simulink model "deng_feng_unpack"  (R2016b)
(part 2 of 28)

      | port_label('input', 1, 'd');
      | port_label('output', 1, 'q');
      | disp(['Z^-', num2str(latency)]);
  pipeline249 : Subsystem  AncestorBlock=casper_library_delays/pipeline  mask(pipeline){latency=2}
      mask help:
      | An explicitly laid-out delay line to avoid mapping to SRL16s
      | for use in pipelining to help achieve timing closure.
      mask init:
      | pipeline_init(gcb,'latency',latency);
      settings: AttributesFormatString=Latency = %<latency>
      mask Display:
      | port_label('input', 1, 'd');
      | port_label('output', 1, 'q');
      | disp(['Z^-', num2str(latency)]);
  pipeline251 : Subsystem  AncestorBlock=casper_library_delays/pipeline  mask(pipeline){latency=2}
      mask help:
      | An explicitly laid-out delay line to avoid mapping to SRL16s
      | for use in pipelining to help achieve timing closure.
      mask init:
      | pipeline_init(gcb,'latency',latency);
      settings: AttributesFormatString=Latency = %<latency>
      mask Display:
      | port_label('input', 1, 'd');
      | port_label('output', 1, 'q');
      | disp(['Z^-', num2str(latency)]);
  pipeline252 : Subsystem  AncestorBlock=casper_library_delays/pipeline  mask(pipeline){latency=2}
      mask help:
      | An explicitly laid-out delay line to avoid mapping to SRL16s
      | for use in pipelining to help achieve timing closure.
      mask init:
      | pipeline_init(gcb,'latency',latency);
      settings: AttributesFormatString=Latency = %<latency>
      mask Display:
      | port_label('input', 1, 'd');
      | port_label('output', 1, 'q');
      | disp(['Z^-', num2str(latency)]);
  pipeline257 : Subsystem  AncestorBlock=casper_library_delays/pipeline  mask(pipeline){latency=2}
      mask help:
      | An explicitly laid-out delay line to avoid mapping to SRL16s
      | for use in pipelining to help achieve timing closure.
      mask init:
      | pipeline_init(gcb,'latency',latency);
      settings: AttributesFormatString=Latency = %<latency>
      mask Display:
      | port_label('input', 1, 'd');
      | port_label('output', 1, 'q');
      | disp(['Z^-', num2str(latency)]);
  pipeline258 : Subsystem  AncestorBlock=casper_library_delays/pipeline  mask(pipeline){latency=2}
      mask help:
      | An explicitly laid-out delay line to avoid mapping to SRL16s
      | for use in pipelining to help achieve timing closure.
      mask init:
      | pipeline_init(gcb,'latency',latency);
      settings: AttributesFormatString=Latency = %<latency>
      mask Display:
      | port_label('input', 1, 'd');
      | port_label('output', 1, 'q');
      | disp(['Z^-', num2str(latency)]);
  pipeline263 : Subsystem  AncestorBlock=casper_library_delays/pipeline  mask(pipeline){latency=2}
      mask help:
      | An explicitly laid-out delay line to avoid mapping to SRL16s
      | for use in pipelining to help achieve timing closure.
      mask init:
      | pipeline_init(gcb,'latency',latency);
      settings: AttributesFormatString=Latency = %<latency>
      mask Display:
      | port_label('input', 1, 'd');
      | port_label('output', 1, 'q');
      | disp(['Z^-', num2str(latency)]);
  pipeline264 : Subsystem  AncestorBlock=casper_library_delays/pipeline  mask(pipeline){latency=2}
      mask help:
      | An explicitly laid-out delay line to avoid mapping to SRL16s
      | for use in pipelining to help achieve timing closure.
      mask init:
      | pipeline_init(gcb,'latency',latency);
      settings: AttributesFormatString=Latency = %<latency>
      mask Display:
      | port_label('input', 1, 'd');
      | port_label('output', 1, 'q');
      | disp(['Z^-', num2str(latency)]);
  pipeline268 : Subsystem  AncestorBlock=casper_library_delays/pipeline  mask(pipeline){latency=2}
      mask help:
      | An explicitly laid-out delay line to avoid mapping to SRL16s
      | for use in pipelining to help achieve timing closure.
      mask init:
      | pipeline_init(gcb,'latency',latency);
      settings: AttributesFormatString=Latency = %<latency>
      mask Display:
      | port_label('input', 1, 'd');
      | port_label('output', 1, 'q');
      | disp(['Z^-', num2str(latency)]);
  pipeline270 : Subsystem  AncestorBlock=casper_library_delays/pipeline  mask(pipeline){latency=1}
      mask help:
      | An explicitly laid-out delay line to avoid mapping to SRL16s
      | for use in pipelining to help achieve timing closure.
      mask init:
      | pipeline_init(gcb,'latency',latency);
      settings: AttributesFormatString=Latency = %<latency>
      mask Display:
      | port_label('input', 1, 'd');
      | port_label('output', 1, 'q');
      | disp(['Z^-', num2str(latency)]);
  pipeline271 : Subsystem  AncestorBlock=casper_library_delays/pipeline  mask(pipeline){latency=2}
      mask help:
      | An explicitly laid-out delay line to avoid mapping to SRL16s
      | for use in pipelining to help achieve timing closure.
      mask init:
      | pipeline_init(gcb,'latency',latency);
      settings: AttributesFormatString=Latency = %<latency>
      mask Display:
      | port_label('input', 1, 'd');
      | port_label('output', 1, 'q');
      | disp(['Z^-', num2str(latency)]);
  pipeline272 : Subsystem  AncestorBlock=casper_library_delays/pipeline  mask(pipeline){latency=2}
      mask help:
      | An explicitly laid-out delay line to avoid mapping to SRL16s
      | for use in pipelining to help achieve timing closure.
      mask init:
      | pipeline_init(gcb,'latency',latency);
      settings: AttributesFormatString=Latency = %<latency>
      mask Display:
      | port_label('input', 1, 'd');
      | port_label('output', 1, 'q');
      | disp(['Z^-', num2str(latency)]);
  pipeline273 : Subsystem  AncestorBlock=casper_library_delays/pipeline  mask(pipeline){latency=2}
      mask help:
      | An explicitly laid-out delay line to avoid mapping to SRL16s
      | for use in pipelining to help achieve timing closure.
      mask init:
      | pipeline_init(gcb,'latency',latency);
      settings: AttributesFormatString=Latency = %<latency>
      mask Display:
      | port_label('input', 1, 'd');
      | port_label('output', 1, 'q');
      | disp(['Z^-', num2str(latency)]);
  pipeline274 : Subsystem  AncestorBlock=casper_library_delays/pipeline  mask(pipeline){latency=2}
      mask help:
      | An explicitly laid-out delay line to avoid mapping to SRL16s
      | for use in pipelining to help achieve timing closure.
      mask init:
      | pipeline_init(gcb,'latency',latency);
      settings: AttributesFormatString=Latency = %<latency>
      mask Display:
      | port_label('input', 1, 'd');
      | port_label('output', 1, 'q');
      | disp(['Z^-', num2str(latency)]);
  pipeline275 : Subsystem  AncestorBlock=casper_library_delays/pipeline  mask(pipeline){latency=2}
      mask help:
      | An explicitly laid-out delay line to avoid mapping to SRL16s
      | for use in pipelining to help achieve timing closure.
      mask init:
      | pipeline_init(gcb,'latency',latency);
      settings: AttributesFormatString=Latency = %<latency>
      mask Display:
      | port_label('input', 1, 'd');
      | port_label('output', 1, 'q');
      | disp(['Z^-', num2str(latency)]);
  pipeline276 : Subsystem  AncestorBlock=casper_library_delays/pipeline  mask(pipeline){latency=2}
      mask help:
      | An explicitly laid-out delay line to avoid mapping to SRL16s
      | for use in pipelining to help achieve timing closure.
      mask init:
      | pipeline_init(gcb,'latency',latency);
      settings: AttributesFormatString=Latency = %<latency>
      mask Display:
      | port_label('input', 1, 'd');
      | port_label('output', 1, 'q');
      | disp(['Z^-', num2str(latency)]);
  pipeline277 : Subsystem  AncestorBlock=casper_library_delays/pipeline  mask(pipeline){latency=2}
      mask help:
      | An explicitly laid-out delay line to avoid mapping to SRL16s
      | for use in pipelining to help achieve timing closure.
      mask init:
      | pipeline_init(gcb,'latency',latency);
      settings: AttributesFormatString=Latency = %<latency>
      mask Display:
      | port_label('input', 1, 'd');
      | port_label('output', 1, 'q');
      | disp(['Z^-', num2str(latency)]);
  pipeline278 : Subsystem  AncestorBlock=casper_library_delays/pipeline  mask(pipeline){latency=2}
      mask help:
      | An explicitly laid-out delay line to avoid mapping to SRL16s
      | for use in pipelining to help achieve timing closure.
      mask init:
      | pipeline_init(gcb,'latency',latency);
      settings: AttributesFormatString=Latency = %<latency>
      mask Display:
      | port_label('input', 1, 'd');
      | port_label('output', 1, 'q');
      | disp(['Z^-', num2str(latency)]);
  pipeline285 : Subsystem  AncestorBlock=casper_library_delays/pipeline  mask(pipeline){latency=2}
      mask help:
      | An explicitly laid-out delay line to avoid mapping to SRL16s
      | for use in pipelining to help achieve timing closure.
      mask init:
      | pipeline_init(gcb,'latency',latency);
      settings: AttributesFormatString=Latency = %<latency>
      mask Display:
      | port_label('input', 1, 'd');
      | port_label('output', 1, 'q');
      | disp(['Z^-', num2str(latency)]);
  pipeline286 : Subsystem  AncestorBlock=casper_library_delays/pipeline  mask(pipeline){latency=2}
      mask help:
      | An explicitly laid-out delay line to avoid mapping to SRL16s
      | for use in pipelining to help achieve timing closure.
      mask init:
      | pipeline_init(gcb,'latency',latency);
      settings: AttributesFormatString=Latency = %<latency>
      mask Display:
      | port_label('input', 1, 'd');
      | port_label('output', 1, 'q');
      | disp(['Z^-', num2str(latency)]);
  pipeline287 : Subsystem  AncestorBlock=casper_library_delays/pipeline  mask(pipeline){latency=2}
      mask help:
      | An explicitly laid-out delay line to avoid mapping to SRL16s
      | for use in pipelining to help achieve timing closure.
      mask init:
      | pipeline_init(gcb,'latency',latency);
      settings: AttributesFormatString=Latency = %<latency>
      mask Display:
      | port_label('input', 1, 'd');
      | port_label('output', 1, 'q');
      | disp(['Z^-', num2str(latency)]);
  pipeline288 : Subsystem  AncestorBlock=casper_library_delays/pipeline  mask(pipeline){latency=2}
      mask help:
      | An explicitly laid-out delay line to avoid mapping to SRL16s
      | for use in pipelining to help achieve timing closure.
      mask init:
      | pipeline_init(gcb,'latency',latency);
      settings: AttributesFormatString=Latency = %<latency>
      mask Display:
      | port_label('input', 1, 'd');
      | port_label('output', 1, 'q');
      | disp(['Z^-', num2str(latency)]);
  pipeline289 : Subsystem  AncestorBlock=casper_library_delays/pipeline  mask(pipeline){latency=2}
      mask help:
      | An explicitly laid-out delay line to avoid mapping to SRL16s
      | for use in pipelining to help achieve timing closure.
      mask init:
      | pipeline_init(gcb,'latency',latency);
      settings: AttributesFormatString=Latency = %<latency>
      mask Display:
      | port_label('input', 1, 'd');
      | port_label('output', 1, 'q');
      | disp(['Z^-', num2str(latency)]);
  pipeline290 : Subsystem  AncestorBlock=casper_library_delays/pipeline  mask(pipeline){latency=2}
      mask help:
      | An explicitly laid-out delay line to avoid mapping to SRL16s
      | for use in pipelining to help achieve timing closure.
      mask init:
      | pipeline_init(gcb,'latency',latency);
      settings: AttributesFormatString=Latency = %<latency>
      mask Display:
      | port_label('input', 1, 'd');
      | port_label('output', 1, 'q');
      | disp(['Z^-', num2str(latency)]);
  pipeline291 : Subsystem  AncestorBlock=casper_library_delays/pipeline  mask(pipeline){latency=2}
      mask help:
      | An explicitly laid-out delay line to avoid mapping to SRL16s
      | for use in pipelining to help achieve timing closure.
      mask init:
      | pipeline_init(gcb,'latency',latency);
      settings: AttributesFormatString=Latency = %<latency>
      mask Display:
      | port_label('input', 1, 'd');
      | port_label('output', 1, 'q');
      | disp(['Z^-', num2str(latency)]);
  pipeline292 : Subsystem  AncestorBlock=casper_library_delays/pipeline  mask(pipeline){latency=2}
      mask help:
      | An explicitly laid-out delay line to avoid mapping to SRL16s
      | for use in pipelining to help achieve timing closure.
      mask init:
      | pipeline_init(gcb,'latency',latency);
      settings: AttributesFormatString=Latency = %<latency>
      mask Display:
      | port_label('input', 1, 'd');
      | port_label('output', 1, 'q');
      | disp(['Z^-', num2str(latency)]);
  pipeline293 : Subsystem  AncestorBlock=casper_library_delays/pipeline  mask(pipeline){latency=2}
      mask help:
      | An explicitly laid-out delay line to avoid mapping to SRL16s
      | for use in pipelining to help achieve timing closure.
      mask init:
      | pipeline_init(gcb,'latency',latency);
      settings: AttributesFormatString=Latency = %<latency>
      mask Display:
      | port_label('input', 1, 'd');
      | port_label('output', 1, 'q');
      | disp(['Z^-', num2str(latency)]);
  pipeline294 : Subsystem  AncestorBlock=casper_library_delays/pipeline  mask(pipeline){latency=2}
      mask help:
      | An explicitly laid-out delay line to avoid mapping to SRL16s
      | for use in pipelining to help achieve timing closure.
      mask init:
      | pipeline_init(gcb,'latency',latency);
      settings: AttributesFormatString=Latency = %<latency>
      mask Display:
      | port_label('input', 1, 'd');
      | port_label('output', 1, 'q');
      | disp(['Z^-', num2str(latency)]);
  pipeline297 : Subsystem  AncestorBlock=casper_library_delays/pipeline  mask(pipeline){latency=2}
      mask help:
      | An explicitly laid-out delay line to avoid mapping to SRL16s
      | for use in pipelining to help achieve timing closure.
      mask init:
      | pipeline_init(gcb,'latency',latency);
      settings: AttributesFormatString=Latency = %<latency>
      mask Display:
      | port_label('input', 1, 'd');
      | port_label('output', 1, 'q');
      | disp(['Z^-', num2str(latency)]);
  pipeline298 : Subsystem  AncestorBlock=casper_library_delays/pipeline  mask(pipeline){latency=2}
      mask help:
      | An explicitly laid-out delay line to avoid mapping to SRL16s
      | for use in pipelining to help achieve timing closure.
      mask init:
      | pipeline_init(gcb,'latency',latency);
      settings: AttributesFormatString=Latency = %<latency>
      mask Display:
      | port_label('input', 1, 'd');
      | port_label('output', 1, 'q');
      | disp(['Z^-', num2str(latency)]);
  pipeline3 : Subsystem  AncestorBlock=casper_library_delays/pipeline  mask(pipeline){latency=2}
      mask help:
      | An explicitly laid-out delay line to avoid mapping to SRL16s
      | for use in pipelining to help achieve timing closure.
      mask init:
      | pipeline_init(gcb,'latency',latency);
      settings: AttributesFormatString=Latency = %<latency>
      mask Display:
      | port_label('input', 1, 'd');
      | port_label('output', 1, 'q');
      | disp(['Z^-', num2str(latency)]);
  pipeline307 : Subsystem  AncestorBlock=casper_library_delays/pipeline  mask(pipeline){latency=2}
      mask help:
      | An explicitly laid-out delay line to avoid mapping to SRL16s
      | for use in pipelining to help achieve timing closure.
      mask init:
      | pipeline_init(gcb,'latency',latency);
      settings: AttributesFormatString=Latency = %<latency>
      mask Display:
      | port_label('input', 1, 'd');
      | port_label('output', 1, 'q');
      | disp(['Z^-', num2str(latency)]);
  pipeline309 : Subsystem  AncestorBlock=casper_library_delays/pipeline  mask(pipeline){latency=2}
      mask help:
      | An explicitly laid-out delay line to avoid mapping to SRL16s
      | for use in pipelining to help achieve timing closure.
      mask init:
      | pipeline_init(gcb,'latency',latency);
      settings: AttributesFormatString=Latency = %<latency>
      mask Display:
      | port_label('input', 1, 'd');
      | port_label('output', 1, 'q');
      | disp(['Z^-', num2str(latency)]);
  pipeline320 : Subsystem  AncestorBlock=casper_library_delays/pipeline  mask(pipeline){latency=2}
      mask help:
      | An explicitly laid-out delay line to avoid mapping to SRL16s
      | for use in pipelining to help achieve timing closure.
      mask init:
      | pipeline_init(gcb,'latency',latency);
      settings: AttributesFormatString=Latency = %<latency>
      mask Display:
      | port_label('input', 1, 'd');
      | port_label('output', 1, 'q');
      | disp(['Z^-', num2str(latency)]);
  pipeline327 : Subsystem  AncestorBlock=casper_library_delays/pipeline  mask(pipeline){latency=2}
      mask help:
      | An explicitly laid-out delay line to avoid mapping to SRL16s
      | for use in pipelining to help achieve timing closure.
      mask init:
      | pipeline_init(gcb,'latency',latency);
      settings: AttributesFormatString=Latency = %<latency>
      mask Display:
      | port_label('input', 1, 'd');
      | port_label('output', 1, 'q');
      | disp(['Z^-', num2str(latency)]);
  pipeline328 : Subsystem  AncestorBlock=casper_library_delays/pipeline  mask(pipeline){latency=2}
      mask help:
      | An explicitly laid-out delay line to avoid mapping to SRL16s
      | for use in pipelining to help achieve timing closure.
      mask init:
      | pipeline_init(gcb,'latency',latency);
      settings: AttributesFormatString=Latency = %<latency>
      mask Display:
      | port_label('input', 1, 'd');
      | port_label('output', 1, 'q');
      | disp(['Z^-', num2str(latency)]);
  pipeline329 : Subsystem  AncestorBlock=casper_library_delays/pipeline  mask(pipeline){latency=2}
      mask help:
      | An explicitly laid-out delay line to avoid mapping to SRL16s
      | for use in pipelining to help achieve timing closure.
      mask init:
      | pipeline_init(gcb,'latency',latency);
      settings: AttributesFormatString=Latency = %<latency>
      mask Display:
      | port_label('input', 1, 'd');
      | port_label('output', 1, 'q');
      | disp(['Z^-', num2str(latency)]);
  pipeline330 : Subsystem  AncestorBlock=casper_library_delays/pipeline  mask(pipeline){latency=2}
      mask help:
      | An explicitly laid-out delay line to avoid mapping to SRL16s
      | for use in pipelining to help achieve timing closure.
      mask init:
      | pipeline_init(gcb,'latency',latency);
      settings: AttributesFormatString=Latency = %<latency>
      mask Display:
      | port_label('input', 1, 'd');
      | port_label('output', 1, 'q');
      | disp(['Z^-', num2str(latency)]);
  pipeline331 : Subsystem  AncestorBlock=casper_library_delays/pipeline  mask(pipeline){latency=2}
      mask help:
      | An explicitly laid-out delay line to avoid mapping to SRL16s
      | for use in pipelining to help achieve timing closure.
      mask init:
      | pipeline_init(gcb,'latency',latency);
      settings: AttributesFormatString=Latency = %<latency>
      mask Display:
      | port_label('input', 1, 'd');
      | port_label('output', 1, 'q');
      | disp(['Z^-', num2str(latency)]);
  pipeline333 : Subsystem  AncestorBlock=casper_library_delays/pipeline  mask(pipeline){latency=2}
      mask help:
      | An explicitly laid-out delay line to avoid mapping to SRL16s
      | for use in pipelining to help achieve timing closure.
      mask init:
      | pipeline_init(gcb,'latency',latency);
      settings: AttributesFormatString=Latency = %<latency>
      mask Display:
      | port_label('input', 1, 'd');
      | port_label('output', 1, 'q');
      | disp(['Z^-', num2str(latency)]);
  pipeline334 : Subsystem  AncestorBlock=casper_library_delays/pipeline  mask(pipeline){latency=2}
      mask help:
      | An explicitly laid-out delay line to avoid mapping to SRL16s
      | for use in pipelining to help achieve timing closure.
      mask init:
      | pipeline_init(gcb,'latency',latency);
      settings: AttributesFormatString=Latency = %<latency>
      mask Display:
      | port_label('input', 1, 'd');
      | port_label('output', 1, 'q');
      | disp(['Z^-', num2str(latency)]);
  pipeline339 : Subsystem  AncestorBlock=casper_library_delays/pipeline  mask(pipeline){latency=2}
      mask help:
      | An explicitly laid-out delay line to avoid mapping to SRL16s
      | for use in pipelining to help achieve timing closure.
      mask init:
      | pipeline_init(gcb,'latency',latency);
      settings: AttributesFormatString=Latency = %<latency>
      mask Display:
      | port_label('input', 1, 'd');
      | port_label('output', 1, 'q');
      | disp(['Z^-', num2str(latency)]);
  pipeline340 : Subsystem  AncestorBlock=casper_library_delays/pipeline  mask(pipeline){latency=2}
      mask help:
      | An explicitly laid-out delay line to avoid mapping to SRL16s
      | for use in pipelining to help achieve timing closure.
      mask init:
      | pipeline_init(gcb,'latency',latency);
      settings: AttributesFormatString=Latency = %<latency>
      mask Display:
      | port_label('input', 1, 'd');
      | port_label('output', 1, 'q');
      | disp(['Z^-', num2str(latency)]);
  pipeline341 : Subsystem  AncestorBlock=casper_library_delays/pipeline  mask(pipeline){latency=2}
      mask help:
      | An explicitly laid-out delay line to avoid mapping to SRL16s
      | for use in pipelining to help achieve timing closure.
      mask init:
      | pipeline_init(gcb,'latency',latency);
      settings: AttributesFormatString=Latency = %<latency>
      mask Display:
      | port_label('input', 1, 'd');
      | port_label('output', 1, 'q');
      | disp(['Z^-', num2str(latency)]);
  pipeline342 : Subsystem  AncestorBlock=casper_library_delays/pipeline  mask(pipeline){latency=2}
      mask help:
      | An explicitly laid-out delay line to avoid mapping to SRL16s
      | for use in pipelining to help achieve timing closure.
      mask init:
      | pipeline_init(gcb,'latency',latency);
      settings: AttributesFormatString=Latency = %<latency>
      mask Display:
      | port_label('input', 1, 'd');
      | port_label('output', 1, 'q');
      | disp(['Z^-', num2str(latency)]);
  pipeline343 : Subsystem  AncestorBlock=casper_library_delays/pipeline  mask(pipeline){latency=2}
      mask help:
      | An explicitly laid-out delay line to avoid mapping to SRL16s
      | for use in pipelining to help achieve timing closure.
      mask init:
      | pipeline_init(gcb,'latency',latency);
      settings: AttributesFormatString=Latency = %<latency>
      mask Display:
      | port_label('input', 1, 'd');
      | port_label('output', 1, 'q');
      | disp(['Z^-', num2str(latency)]);
  pipeline344 : Subsystem  AncestorBlock=casper_library_delays/pipeline  mask(pipeline){latency=2}
      mask help:
      | An explicitly laid-out delay line to avoid mapping to SRL16s
      | for use in pipelining to help achieve timing closure.
      mask init:
      | pipeline_init(gcb,'latency',latency);
      settings: AttributesFormatString=Latency = %<latency>
      mask Display:
      | port_label('input', 1, 'd');
      | port_label('output', 1, 'q');
      | disp(['Z^-', num2str(latency)]);
  pipeline345 : Subsystem  AncestorBlock=casper_library_delays/pipeline  mask(pipeline){latency=2}
      mask help:
      | An explicitly laid-out delay line to avoid mapping to SRL16s
      | for use in pipelining to help achieve timing closure.
      mask init:
      | pipeline_init(gcb,'latency',latency);
      settings: AttributesFormatString=Latency = %<latency>
      mask Display:
      | port_label('input', 1, 'd');
      | port_label('output', 1, 'q');
      | disp(['Z^-', num2str(latency)]);
  pipeline346 : Subsystem  AncestorBlock=casper_library_delays/pipeline  mask(pipeline){latency=2}
      mask help:
      | An explicitly laid-out delay line to avoid mapping to SRL16s
      | for use in pipelining to help achieve timing closure.
      mask init:
      | pipeline_init(gcb,'latency',latency);
      settings: AttributesFormatString=Latency = %<latency>
      mask Display:
      | port_label('input', 1, 'd');
      | port_label('output', 1, 'q');
      | disp(['Z^-', num2str(latency)]);
  pipeline347 : Subsystem  AncestorBlock=casper_library_delays/pipeline  mask(pipeline){latency=2}
      mask help:
      | An explicitly laid-out delay line to avoid mapping to SRL16s
      | for use in pipelining to help achieve timing closure.
      mask init:
      | pipeline_init(gcb,'latency',latency);
      settings: AttributesFormatString=Latency = %<latency>
      mask Display:
      | port_label('input', 1, 'd');
      | port_label('output', 1, 'q');
      | disp(['Z^-', num2str(latency)]);
  pipeline348 : Subsystem  AncestorBlock=casper_library_delays/pipeline  mask(pipeline){latency=2}
      mask help:
      | An explicitly laid-out delay line to avoid mapping to SRL16s
      | for use in pipelining to help achieve timing closure.
      mask init:
      | pipeline_init(gcb,'latency',latency);
      settings: AttributesFormatString=Latency = %<latency>
      mask Display:
      | port_label('input', 1, 'd');
      | port_label('output', 1, 'q');
      | disp(['Z^-', num2str(latency)]);
  pipeline349 : Subsystem  AncestorBlock=casper_library_delays/pipeline  mask(pipeline){latency=2}
      mask help:
      | An explicitly laid-out delay line to avoid mapping to SRL16s
      | for use in pipelining to help achieve timing closure.
      mask init:
      | pipeline_init(gcb,'latency',latency);
      settings: AttributesFormatString=Latency = %<latency>
      mask Display:
      | port_label('input', 1, 'd');
      | port_label('output', 1, 'q');
      | disp(['Z^-', num2str(latency)]);
  pipeline350 : Subsystem  AncestorBlock=casper_library_delays/pipeline  mask(pipeline){latency=2}
      mask help:
      | An explicitly laid-out delay line to avoid mapping to SRL16s
      | for use in pipelining to help achieve timing closure.
      mask init:
      | pipeline_init(gcb,'latency',latency);
      settings: AttributesFormatString=Latency = %<latency>
      mask Display:
      | port_label('input', 1, 'd');
      | port_label('output', 1, 'q');
      | disp(['Z^-', num2str(latency)]);
  pipeline351 : Subsystem  AncestorBlock=casper_library_delays/pipeline  mask(pipeline){latency=2}
      mask help:
      | An explicitly laid-out delay line to avoid mapping to SRL16s
      | for use in pipelining to help achieve timing closure.
      mask init:
      | pipeline_init(gcb,'latency',latency);
      settings: AttributesFormatString=Latency = %<latency>
      mask Display:
      | port_label('input', 1, 'd');
      | port_label('output', 1, 'q');
      | disp(['Z^-', num2str(latency)]);
  pipeline352 : Subsystem  AncestorBlock=casper_library_delays/pipeline  mask(pipeline){latency=2}
      mask help:
      | An explicitly laid-out delay line to avoid mapping to SRL16s
      | for use in pipelining to help achieve timing closure.
      mask init:
      | pipeline_init(gcb,'latency',latency);
      settings: AttributesFormatString=Latency = %<latency>
      mask Display:
      | port_label('input', 1, 'd');
      | port_label('output', 1, 'q');
      | disp(['Z^-', num2str(latency)]);
  pipeline353 : Subsystem  AncestorBlock=casper_library_delays/pipeline  mask(pipeline){latency=1}
      mask help:
      | An explicitly laid-out delay line to avoid mapping to SRL16s
      | for use in pipelining to help achieve timing closure.
      mask init:
      | pipeline_init(gcb,'latency',latency);
      settings: AttributesFormatString=Latency = %<latency>
      mask Display:
      | port_label('input', 1, 'd');
      | port_label('output', 1, 'q');
      | disp(['Z^-', num2str(latency)]);
  pipeline354 : Subsystem  AncestorBlock=casper_library_delays/pipeline  mask(pipeline){latency=1}
      mask help:
      | An explicitly laid-out delay line to avoid mapping to SRL16s
      | for use in pipelining to help achieve timing closure.
      mask init:
      | pipeline_init(gcb,'latency',latency);
      settings: AttributesFormatString=Latency = %<latency>
      mask Display:
      | port_label('input', 1, 'd');
      | port_label('output', 1, 'q');
      | disp(['Z^-', num2str(latency)]);
  pipeline355 : Subsystem  AncestorBlock=casper_library_delays/pipeline  mask(pipeline){latency=1}
      mask help:
      | An explicitly laid-out delay line to avoid mapping to SRL16s
      | for use in pipelining to help achieve timing closure.
      mask init:
      | pipeline_init(gcb,'latency',latency);
      settings: AttributesFormatString=Latency = %<latency>
      mask Display:
      | port_label('input', 1, 'd');
      | port_label('output', 1, 'q');
      | disp(['Z^-', num2str(latency)]);
  pipeline356 : Subsystem  AncestorBlock=casper_library_delays/pipeline  mask(pipeline){latency=3}
      mask help:
      | An explicitly laid-out delay line to avoid mapping to SRL16s
      | for use in pipelining to help achieve timing closure.
      mask init:
      | pipeline_init(gcb,'latency',latency);
      settings: AttributesFormatString=Latency = %<latency>
      mask Display:
      | port_label('input', 1, 'd');
      | port_label('output', 1, 'q');
      | disp(['Z^-', num2str(latency)]);
  pipeline361 : Subsystem  AncestorBlock=casper_library_delays/pipeline  mask(pipeline){latency=2}
      mask help:
      | An explicitly laid-out delay line to avoid mapping to SRL16s
      | for use in pipelining to help achieve timing closure.
      mask init:
      | pipeline_init(gcb,'latency',latency);
      settings: AttributesFormatString=Latency = %<latency>
      mask Display:
      | port_label('input', 1, 'd');
      | port_label('output', 1, 'q');
      | disp(['Z^-', num2str(latency)]);
  pipeline364 : Subsystem  AncestorBlock=casper_library_delays/pipeline  mask(pipeline){latency=1}
      mask help:
      | An explicitly laid-out delay line to avoid mapping to SRL16s
      | for use in pipelining to help achieve timing closure.
      mask init:
      | pipeline_init(gcb,'latency',latency);
      settings: AttributesFormatString=Latency = %<latency>
      mask Display:
      | port_label('input', 1, 'd');
      | port_label('output', 1, 'q');
      | disp(['Z^-', num2str(latency)]);
  pipeline365 : Subsystem  AncestorBlock=casper_library_delays/pipeline  mask(pipeline){latency=1}
      mask help:
      | An explicitly laid-out delay line to avoid mapping to SRL16s
      | for use in pipelining to help achieve timing closure.
      mask init:
      | pipeline_init(gcb,'latency',latency);
      settings: AttributesFormatString=Latency = %<latency>
      mask Display:
      | port_label('input', 1, 'd');
      | port_label('output', 1, 'q');
      | disp(['Z^-', num2str(latency)]);
  pipeline366 : Subsystem  AncestorBlock=casper_library_delays/pipeline  mask(pipeline){latency=1}
      mask help:
      | An explicitly laid-out delay line to avoid mapping to SRL16s
      | for use in pipelining to help achieve timing closure.
      mask init:
      | pipeline_init(gcb,'latency',latency);
      settings: AttributesFormatString=Latency = %<latency>
      mask Display:
      | port_label('input', 1, 'd');
      | port_label('output', 1, 'q');
      | disp(['Z^-', num2str(latency)]);
  pipeline367 : Subsystem  AncestorBlock=casper_library_delays/pipeline  mask(pipeline){latency=1}
      mask help:
      | An explicitly laid-out delay line to avoid mapping to SRL16s
      | for use in pipelining to help achieve timing closure.
      mask init:
      | pipeline_init(gcb,'latency',latency);
      settings: AttributesFormatString=Latency = %<latency>
      mask Display:
      | port_label('input', 1, 'd');
      | port_label('output', 1, 'q');
      | disp(['Z^-', num2str(latency)]);
  pipeline368 : Subsystem  AncestorBlock=casper_library_delays/pipeline  mask(pipeline){latency=1}
      mask help:
      | An explicitly laid-out delay line to avoid mapping to SRL16s
      | for use in pipelining to help achieve timing closure.
      mask init:
      | pipeline_init(gcb,'latency',latency);
      settings: AttributesFormatString=Latency = %<latency>
      mask Display:
      | port_label('input', 1, 'd');
      | port_label('output', 1, 'q');
      | disp(['Z^-', num2str(latency)]);
  pipeline369 : Subsystem  AncestorBlock=casper_library_delays/pipeline  mask(pipeline){latency=3}
      mask help:
      | An explicitly laid-out delay line to avoid mapping to SRL16s
      | for use in pipelining to help achieve timing closure.
      mask init:
      | pipeline_init(gcb,'latency',latency);
      settings: AttributesFormatString=Latency = %<latency>
      mask Display:
      | port_label('input', 1, 'd');
      | port_label('output', 1, 'q');
      | disp(['Z^-', num2str(latency)]);
  pipeline370 : Subsystem  AncestorBlock=casper_library_delays/pipeline  mask(pipeline){latency=1}
      mask help:
      | An explicitly laid-out delay line to avoid mapping to SRL16s
      | for use in pipelining to help achieve timing closure.
      mask init:
      | pipeline_init(gcb,'latency',latency);
      settings: AttributesFormatString=Latency = %<latency>
      mask Display:
      | port_label('input', 1, 'd');
      | port_label('output', 1, 'q');
      | disp(['Z^-', num2str(latency)]);
  pipeline371 : Subsystem  AncestorBlock=casper_library_delays/pipeline  mask(pipeline){latency=1}
      mask help:
      | An explicitly laid-out delay line to avoid mapping to SRL16s
      | for use in pipelining to help achieve timing closure.
      mask init:
      | pipeline_init(gcb,'latency',latency);
      settings: AttributesFormatString=Latency = %<latency>
      mask Display:
      | port_label('input', 1, 'd');
      | port_label('output', 1, 'q');
      | disp(['Z^-', num2str(latency)]);
  pipeline372 : Subsystem  AncestorBlock=casper_library_delays/pipeline  mask(pipeline){latency=2}
      mask help:
      | An explicitly laid-out delay line to avoid mapping to SRL16s
      | for use in pipelining to help achieve timing closure.
      mask init:
      | pipeline_init(gcb,'latency',latency);
      settings: AttributesFormatString=Latency = %<latency>
      mask Display:
      | port_label('input', 1, 'd');
      | port_label('output', 1, 'q');
      | disp(['Z^-', num2str(latency)]);
  pipeline373 : Subsystem  AncestorBlock=casper_library_delays/pipeline  mask(pipeline){latency=1}
      mask help:
      | An explicitly laid-out delay line to avoid mapping to SRL16s
      | for use in pipelining to help achieve timing closure.
      mask init:
      | pipeline_init(gcb,'latency',latency);
      settings: AttributesFormatString=Latency = %<latency>
      mask Display:
      | port_label('input', 1, 'd');
      | port_label('output', 1, 'q');
      | disp(['Z^-', num2str(latency)]);
  pipeline374 : Subsystem  AncestorBlock=casper_library_delays/pipeline  mask(pipeline){latency=1}
      mask help:
      | An explicitly laid-out delay line to avoid mapping to SRL16s
      | for use in pipelining to help achieve timing closure.
      mask init:
      | pipeline_init(gcb,'latency',latency);
      settings: AttributesFormatString=Latency = %<latency>
      mask Display:
      | port_label('input', 1, 'd');
      | port_label('output', 1, 'q');
      | disp(['Z^-', num2str(latency)]);
  pipeline375 : Subsystem  AncestorBlock=casper_library_delays/pipeline  mask(pipeline){latency=1}
      mask help:
      | An explicitly laid-out delay line to avoid mapping to SRL16s
      | for use in pipelining to help achieve timing closure.
      mask init:
      | pipeline_init(gcb,'latency',latency);
      settings: AttributesFormatString=Latency = %<latency>
      mask Display:
      | port_label('input', 1, 'd');
      | port_label('output', 1, 'q');
      | disp(['Z^-', num2str(latency)]);
  pipeline376 : Subsystem  AncestorBlock=casper_library_delays/pipeline  mask(pipeline){latency=3}
      mask help:
      | An explicitly laid-out delay line to avoid mapping to SRL16s
      | for use in pipelining to help achieve timing closure.
      mask init:
      | pipeline_init(gcb,'latency',latency);
      settings: AttributesFormatString=Latency = %<latency>
      mask Display:
      | port_label('input', 1, 'd');
      | port_label('output', 1, 'q');
      | disp(['Z^-', num2str(latency)]);
  pipeline377 : Subsystem  AncestorBlock=casper_library_delays/pipeline  mask(pipeline){latency=1}
      mask help:
      | An explicitly laid-out delay line to avoid mapping to SRL16s
      | for use in pipelining to help achieve timing closure.
      mask init:
      | pipeline_init(gcb,'latency',latency);
      settings: AttributesFormatString=Latency = %<latency>
      mask Display:
      | port_label('input', 1, 'd');
      | port_label('output', 1, 'q');
      | disp(['Z^-', num2str(latency)]);
  pipeline378 : Subsystem  AncestorBlock=casper_library_delays/pipeline  mask(pipeline){latency=1}
      mask help:
      | An explicitly laid-out delay line to avoid mapping to SRL16s
      | for use in pipelining to help achieve timing closure.
      mask init:
      | pipeline_init(gcb,'latency',latency);
      settings: AttributesFormatString=Latency = %<latency>
      mask Display:
      | port_label('input', 1, 'd');
      | port_label('output', 1, 'q');
      | disp(['Z^-', num2str(latency)]);
  pipeline379 : Subsystem  AncestorBlock=casper_library_delays/pipeline  mask(pipeline){latency=3}
      mask help:
      | An explicitly laid-out delay line to avoid mapping to SRL16s
      | for use in pipelining to help achieve timing closure.
      mask init:
      | pipeline_init(gcb,'latency',latency);
      settings: AttributesFormatString=Latency = %<latency>
      mask Display:
      | port_label('input', 1, 'd');
      | port_label('output', 1, 'q');
      | disp(['Z^-', num2str(latency)]);
  pipeline38 : Subsystem  AncestorBlock=casper_library_delays/pipeline  mask(pipeline){latency=2}
      mask help:
      | An explicitly laid-out delay line to avoid mapping to SRL16s
      | for use in pipelining to help achieve timing closure.
      mask init:
      | pipeline_init(gcb,'latency',latency);
      settings: AttributesFormatString=Latency = %<latency>
      mask Display:
      | port_label('input', 1, 'd');
      | port_label('output', 1, 'q');
      | disp(['Z^-', num2str(latency)]);
  pipeline380 : Subsystem  AncestorBlock=casper_library_delays/pipeline  mask(pipeline){latency=3}
      mask help:
      | An explicitly laid-out delay line to avoid mapping to SRL16s
      | for use in pipelining to help achieve timing closure.
      mask init:
      | pipeline_init(gcb,'latency',latency);
      settings: AttributesFormatString=Latency = %<latency>
      mask Display:
      | port_label('input', 1, 'd');
      | port_label('output', 1, 'q');
      | disp(['Z^-', num2str(latency)]);
  pipeline381 : Subsystem  AncestorBlock=casper_library_delays/pipeline  mask(pipeline){latency=3}
      mask help:
      | An explicitly laid-out delay line to avoid mapping to SRL16s
      | for use in pipelining to help achieve timing closure.
      mask init:
      | pipeline_init(gcb,'latency',latency);
      settings: AttributesFormatString=Latency = %<latency>
      mask Display:
      | port_label('input', 1, 'd');
      | port_label('output', 1, 'q');
      | disp(['Z^-', num2str(latency)]);
  pipeline382 : Subsystem  AncestorBlock=casper_library_delays/pipeline  mask(pipeline){latency=3}
      mask help:
      | An explicitly laid-out delay line to avoid mapping to SRL16s
      | for use in pipelining to help achieve timing closure.
      mask init:
      | pipeline_init(gcb,'latency',latency);
      settings: AttributesFormatString=Latency = %<latency>
      mask Display:
      | port_label('input', 1, 'd');
      | port_label('output', 1, 'q');
      | disp(['Z^-', num2str(latency)]);
  pipeline383 : Subsystem  AncestorBlock=casper_library_delays/pipeline  mask(pipeline){latency=2}
      mask help:
      | An explicitly laid-out delay line to avoid mapping to SRL16s
      | for use in pipelining to help achieve timing closure.
      mask init:
      | pipeline_init(gcb,'latency',latency);
      settings: AttributesFormatString=Latency = %<latency>
      mask Display:
      | port_label('input', 1, 'd');
      | port_label('output', 1, 'q');
      | disp(['Z^-', num2str(latency)]);
  pipeline384 : Subsystem  AncestorBlock=casper_library_delays/pipeline  mask(pipeline){latency=3}
      mask help:
      | An explicitly laid-out delay line to avoid mapping to SRL16s
      | for use in pipelining to help achieve timing closure.
      mask init:
      | pipeline_init(gcb,'latency',latency);
      settings: AttributesFormatString=Latency = %<latency>
      mask Display:
      | port_label('input', 1, 'd');
      | port_label('output', 1, 'q');
      | disp(['Z^-', num2str(latency)]);
  pipeline385 : Subsystem  AncestorBlock=casper_library_delays/pipeline  mask(pipeline){latency=3}
      mask help:
      | An explicitly laid-out delay line to avoid mapping to SRL16s
      | for use in pipelining to help achieve timing closure.
      mask init:
      | pipeline_init(gcb,'latency',latency);
      settings: AttributesFormatString=Latency = %<latency>
      mask Display:
      | port_label('input', 1, 'd');
      | port_label('output', 1, 'q');
      | disp(['Z^-', num2str(latency)]);
  pipeline386 : Subsystem  AncestorBlock=casper_library_delays/pipeline  mask(pipeline){latency=3}
      mask help:
      | An explicitly laid-out delay line to avoid mapping to SRL16s
      | for use in pipelining to help achieve timing closure.
      mask init:
      | pipeline_init(gcb,'latency',latency);
      settings: AttributesFormatString=Latency = %<latency>
      mask Display:
      | port_label('input', 1, 'd');
      | port_label('output', 1, 'q');
      | disp(['Z^-', num2str(latency)]);
  pipeline387 : Subsystem  AncestorBlock=casper_library_delays/pipeline  mask(pipeline){latency=3}
      mask help:
      | An explicitly laid-out delay line to avoid mapping to SRL16s
      | for use in pipelining to help achieve timing closure.
      mask init:
      | pipeline_init(gcb,'latency',latency);
      settings: AttributesFormatString=Latency = %<latency>
      mask Display:
      | port_label('input', 1, 'd');
      | port_label('output', 1, 'q');
      | disp(['Z^-', num2str(latency)]);
  pipeline388 : Subsystem  AncestorBlock=casper_library_delays/pipeline  mask(pipeline){latency=3}
      mask help:
      | An explicitly laid-out delay line to avoid mapping to SRL16s
      | for use in pipelining to help achieve timing closure.
      mask init:
      | pipeline_init(gcb,'latency',latency);
      settings: AttributesFormatString=Latency = %<latency>
      mask Display:
      | port_label('input', 1, 'd');
      | port_label('output', 1, 'q');
      | disp(['Z^-', num2str(latency)]);
  pipeline389 : Subsystem  AncestorBlock=casper_library_delays/pipeline  mask(pipeline){latency=2}
      mask help:
      | An explicitly laid-out delay line to avoid mapping to SRL16s
      | for use in pipelining to help achieve timing closure.
      mask init:
      | pipeline_init(gcb,'latency',latency);
      settings: AttributesFormatString=Latency = %<latency>
      mask Display:
      | port_label('input', 1, 'd');
      | port_label('output', 1, 'q');
      | disp(['Z^-', num2str(latency)]);
  pipeline39 : Subsystem  AncestorBlock=casper_library_delays/pipeline  mask(pipeline){latency=2}
      mask help:
      | An explicitly laid-out delay line to avoid mapping to SRL16s
      | for use in pipelining to help achieve timing closure.
      mask init:
      | pipeline_init(gcb,'latency',latency);
      settings: AttributesFormatString=Latency = %<latency>
      mask Display:
      | port_label('input', 1, 'd');
      | port_label('output', 1, 'q');
      | disp(['Z^-', num2str(latency)]);
  pipeline390 : Subsystem  AncestorBlock=casper_library_delays/pipeline  mask(pipeline){latency=2}
      mask help:
      | An explicitly laid-out delay line to avoid mapping to SRL16s
      | for use in pipelining to help achieve timing closure.
      mask init:
      | pipeline_init(gcb,'latency',latency);
      settings: AttributesFormatString=Latency = %<latency>
      mask Display:
      | port_label('input', 1, 'd');
      | port_label('output', 1, 'q');
      | disp(['Z^-', num2str(latency)]);
  pipeline391 : Subsystem  AncestorBlock=casper_library_delays/pipeline  mask(pipeline){latency=2}
      mask help:
      | An explicitly laid-out delay line to avoid mapping to SRL16s
      | for use in pipelining to help achieve timing closure.
      mask init:
      | pipeline_init(gcb,'latency',latency);
      settings: AttributesFormatString=Latency = %<latency>
      mask Display:
      | port_label('input', 1, 'd');
      | port_label('output', 1, 'q');
      | disp(['Z^-', num2str(latency)]);
  pipeline392 : Subsystem  AncestorBlock=casper_library_delays/pipeline  mask(pipeline){latency=2}
      mask help:
      | An explicitly laid-out delay line to avoid mapping to SRL16s
      | for use in pipelining to help achieve timing closure.
      mask init:
      | pipeline_init(gcb,'latency',latency);
      settings: AttributesFormatString=Latency = %<latency>
      mask Display:
      | port_label('input', 1, 'd');
      | port_label('output', 1, 'q');
      | disp(['Z^-', num2str(latency)]);
  pipeline393 : Subsystem  AncestorBlock=casper_library_delays/pipeline  mask(pipeline){latency=2}
      mask help:
      | An explicitly laid-out delay line to avoid mapping to SRL16s
      | for use in pipelining to help achieve timing closure.
      mask init:
      | pipeline_init(gcb,'latency',latency);
      settings: AttributesFormatString=Latency = %<latency>
      mask Display:
      | port_label('input', 1, 'd');
      | port_label('output', 1, 'q');
      | disp(['Z^-', num2str(latency)]);
  pipeline394 : Subsystem  AncestorBlock=casper_library_delays/pipeline  mask(pipeline){latency=2}
      mask help:
      | An explicitly laid-out delay line to avoid mapping to SRL16s
      | for use in pipelining to help achieve timing closure.
      mask init:
      | pipeline_init(gcb,'latency',latency);
      settings: AttributesFormatString=Latency = %<latency>
      mask Display:
      | port_label('input', 1, 'd');
      | port_label('output', 1, 'q');
      | disp(['Z^-', num2str(latency)]);
  pipeline395 : Subsystem  AncestorBlock=casper_library_delays/pipeline  mask(pipeline){latency=2}
      mask help:
      | An explicitly laid-out delay line to avoid mapping to SRL16s
      | for use in pipelining to help achieve timing closure.
      mask init:
      | pipeline_init(gcb,'latency',latency);
      settings: AttributesFormatString=Latency = %<latency>
      mask Display:
      | port_label('input', 1, 'd');
      | port_label('output', 1, 'q');
      | disp(['Z^-', num2str(latency)]);
  pipeline396 : Subsystem  AncestorBlock=casper_library_delays/pipeline  mask(pipeline){latency=2}
      mask help:
      | An explicitly laid-out delay line to avoid mapping to SRL16s
      | for use in pipelining to help achieve timing closure.
      mask init:
      | pipeline_init(gcb,'latency',latency);
      settings: AttributesFormatString=Latency = %<latency>
      mask Display:
      | port_label('input', 1, 'd');
      | port_label('output', 1, 'q');
      | disp(['Z^-', num2str(latency)]);
  pipeline397 : Subsystem  AncestorBlock=casper_library_delays/pipeline  mask(pipeline){latency=2}
      mask help:
      | An explicitly laid-out delay line to avoid mapping to SRL16s
      | for use in pipelining to help achieve timing closure.
      mask init:
      | pipeline_init(gcb,'latency',latency);
      settings: AttributesFormatString=Latency = %<latency>
      mask Display:
      | port_label('input', 1, 'd');
      | port_label('output', 1, 'q');
      | disp(['Z^-', num2str(latency)]);
  pipeline398 : Subsystem  AncestorBlock=casper_library_delays/pipeline  mask(pipeline){latency=2}
      mask help:
      | An explicitly laid-out delay line to avoid mapping to SRL16s
      | for use in pipelining to help achieve timing closure.
      mask init:
      | pipeline_init(gcb,'latency',latency);
      settings: AttributesFormatString=Latency = %<latency>
      mask Display:
      | port_label('input', 1, 'd');
      | port_label('output', 1, 'q');
      | disp(['Z^-', num2str(latency)]);
  pipeline399 : Subsystem  AncestorBlock=casper_library_delays/pipeline  mask(pipeline){latency=2}
      mask help:
      | An explicitly laid-out delay line to avoid mapping to SRL16s
      | for use in pipelining to help achieve timing closure.
      mask init:
      | pipeline_init(gcb,'latency',latency);
      settings: AttributesFormatString=Latency = %<latency>
      mask Display:
      | port_label('input', 1, 'd');
      | port_label('output', 1, 'q');
      | disp(['Z^-', num2str(latency)]);
  pipeline400 : Subsystem  AncestorBlock=casper_library_delays/pipeline  mask(pipeline){latency=2}
      mask help:
      | An explicitly laid-out delay line to avoid mapping to SRL16s
      | for use in pipelining to help achieve timing closure.
      mask init:
      | pipeline_init(gcb,'latency',latency);
      settings: AttributesFormatString=Latency = %<latency>
      mask Display:
      | port_label('input', 1, 'd');
      | port_label('output', 1, 'q');
      | disp(['Z^-', num2str(latency)]);
  pipeline401 : Subsystem  AncestorBlock=casper_library_delays/pipeline  mask(pipeline){latency=2}
      mask help:
      | An explicitly laid-out delay line to avoid mapping to SRL16s
      | for use in pipelining to help achieve timing closure.
      mask init:
      | pipeline_init(gcb,'latency',latency);
      settings: AttributesFormatString=Latency = %<latency>
      mask Display:
      | port_label('input', 1, 'd');
      | port_label('output', 1, 'q');
      | disp(['Z^-', num2str(latency)]);
  pipeline402 : Subsystem  AncestorBlock=casper_library_delays/pipeline  mask(pipeline){latency=2}
      mask help:
      | An explicitly laid-out delay line to avoid mapping to SRL16s
      | for use in pipelining to help achieve timing closure.
      mask init:
      | pipeline_init(gcb,'latency',latency);
      settings: AttributesFormatString=Latency = %<latency>
      mask Display:
      | port_label('input', 1, 'd');
      | port_label('output', 1, 'q');
      | disp(['Z^-', num2str(latency)]);
  pipeline403 : Subsystem  AncestorBlock=casper_library_delays/pipeline  mask(pipeline){latency=2}
      mask help:
      | An explicitly laid-out delay line to avoid mapping to SRL16s
      | for use in pipelining to help achieve timing closure.
      mask init:
      | pipeline_init(gcb,'latency',latency);
      settings: AttributesFormatString=Latency = %<latency>
      mask Display:
      | port_label('input', 1, 'd');
      | port_label('output', 1, 'q');
      | disp(['Z^-', num2str(latency)]);
  pipeline404 : Subsystem  AncestorBlock=casper_library_delays/pipeline  mask(pipeline){latency=2}
      mask help:
      | An explicitly laid-out delay line to avoid mapping to SRL16s
      | for use in pipelining to help achieve timing closure.
      mask init:
      | pipeline_init(gcb,'latency',latency);
      settings: AttributesFormatString=Latency = %<latency>
      mask Display:
      | port_label('input', 1, 'd');
      | port_label('output', 1, 'q');
      | disp(['Z^-', num2str(latency)]);
  pipeline405 : Subsystem  AncestorBlock=casper_library_delays/pipeline  mask(pipeline){latency=2}
      mask help:
      | An explicitly laid-out delay line to avoid mapping to SRL16s
      | for use in pipelining to help achieve timing closure.
      mask init:
      | pipeline_init(gcb,'latency',latency);
      settings: AttributesFormatString=Latency = %<latency>
      mask Display:
      | port_label('input', 1, 'd');
      | port_label('output', 1, 'q');
      | disp(['Z^-', num2str(latency)]);
  pipeline406 : Subsystem  AncestorBlock=casper_library_delays/pipeline  mask(pipeline){latency=2}
      mask help:
      | An explicitly laid-out delay line to avoid mapping to SRL16s
      | for use in pipelining to help achieve timing closure.
      mask init:
      | pipeline_init(gcb,'latency',latency);
      settings: AttributesFormatString=Latency = %<latency>
      mask Display:
      | port_label('input', 1, 'd');
      | port_label('output', 1, 'q');
      | disp(['Z^-', num2str(latency)]);
  pipeline410 : Subsystem  AncestorBlock=casper_library_delays/pipeline  mask(pipeline){latency=2}
      mask help:
      | An explicitly laid-out delay line to avoid mapping to SRL16s
      | for use in pipelining to help achieve timing closure.
      mask init:
      | pipeline_init(gcb,'latency',latency);
      settings: AttributesFormatString=Latency = %<latency>
      mask Display:
      | port_label('input', 1, 'd');
      | port_label('output', 1, 'q');
      | disp(['Z^-', num2str(latency)]);
  pipeline411 : Subsystem  AncestorBlock=casper_library_delays/pipeline  mask(pipeline){latency=2}
      mask help:
      | An explicitly laid-out delay line to avoid mapping to SRL16s
      | for use in pipelining to help achieve timing closure.
      mask init:
      | pipeline_init(gcb,'latency',latency);
      settings: AttributesFormatString=Latency = %<latency>
      mask Display:
      | port_label('input', 1, 'd');
      | port_label('output', 1, 'q');
      | disp(['Z^-', num2str(latency)]);
  pipeline416 : Subsystem  AncestorBlock=casper_library_delays/pipeline  mask(pipeline){latency=2}
      mask help:
      | An explicitly laid-out delay line to avoid mapping to SRL16s
      | for use in pipelining to help achieve timing closure.
      mask init:
      | pipeline_init(gcb,'latency',latency);
      settings: AttributesFormatString=Latency = %<latency>
      mask Display:
      | port_label('input', 1, 'd');
      | port_label('output', 1, 'q');
      | disp(['Z^-', num2str(latency)]);
  pipeline417 : Subsystem  AncestorBlock=casper_library_delays/pipeline  mask(pipeline){latency=2}
      mask help:
      | An explicitly laid-out delay line to avoid mapping to SRL16s
      | for use in pipelining to help achieve timing closure.
      mask init:
      | pipeline_init(gcb,'latency',latency);
      settings: AttributesFormatString=Latency = %<latency>
      mask Display:
      | port_label('input', 1, 'd');
      | port_label('output', 1, 'q');
      | disp(['Z^-', num2str(latency)]);
  pipeline418 : Subsystem  AncestorBlock=casper_library_delays/pipeline  mask(pipeline){latency=2}
      mask help:
      | An explicitly laid-out delay line to avoid mapping to SRL16s
      | for use in pipelining to help achieve timing closure.
      mask init:
      | pipeline_init(gcb,'latency',latency);
      settings: AttributesFormatString=Latency = %<latency>
      mask Display:
      | port_label('input', 1, 'd');
      | port_label('output', 1, 'q');
      | disp(['Z^-', num2str(latency)]);
  pipeline421 : Subsystem  AncestorBlock=casper_library_delays/pipeline  mask(pipeline){latency=3}
      mask help:
      | An explicitly laid-out delay line to avoid mapping to SRL16s
      | for use in pipelining to help achieve timing closure.
      mask init:
      | pipeline_init(gcb,'latency',latency);
      settings: AttributesFormatString=Latency = %<latency>
      mask Display:
      | port_label('input', 1, 'd');
      | port_label('output', 1, 'q');
      | disp(['Z^-', num2str(latency)]);
  pipeline422 : Subsystem  AncestorBlock=casper_library_delays/pipeline  mask(pipeline){latency=6}
      mask help:
      | An explicitly laid-out delay line to avoid mapping to SRL16s
      | for use in pipelining to help achieve timing closure.
      mask init:
      | pipeline_init(gcb,'latency',latency);
      settings: AttributesFormatString=Latency = %<latency>
      mask Display:
      | port_label('input', 1, 'd');
      | port_label('output', 1, 'q');
      | disp(['Z^-', num2str(latency)]);
  pipeline424 : Subsystem  AncestorBlock=casper_library_delays/pipeline  mask(pipeline){latency=2}
      mask help:
      | An explicitly laid-out delay line to avoid mapping to SRL16s
      | for use in pipelining to help achieve timing closure.
      mask init:
      | pipeline_init(gcb,'latency',latency);
      settings: AttributesFormatString=Latency = %<latency>
      mask Display:
      | port_label('input', 1, 'd');
      | port_label('output', 1, 'q');
      | disp(['Z^-', num2str(latency)]);
  pipeline43 : Subsystem  AncestorBlock=casper_library_delays/pipeline  mask(pipeline){latency=2}
      mask help:
      | An explicitly laid-out delay line to avoid mapping to SRL16s
      | for use in pipelining to help achieve timing closure.
      mask init:
      | pipeline_init(gcb,'latency',latency);
      settings: AttributesFormatString=Latency = %<latency>
      mask Display:
      | port_label('input', 1, 'd');
      | port_label('output', 1, 'q');
      | disp(['Z^-', num2str(latency)]);
  pipeline430 : Subsystem  AncestorBlock=casper_library_delays/pipeline  mask(pipeline){latency=2}
      mask help:
      | An explicitly laid-out delay line to avoid mapping to SRL16s
      | for use in pipelining to help achieve timing closure.
      mask init:
      | pipeline_init(gcb,'latency',latency);
      settings: AttributesFormatString=Latency = %<latency>
      mask Display:
      | port_label('input', 1, 'd');
      | port_label('output', 1, 'q');
      | disp(['Z^-', num2str(latency)]);
  pipeline431 : Subsystem  AncestorBlock=casper_library_delays/pipeline  mask(pipeline){latency=2}
      mask help:
      | An explicitly laid-out delay line to avoid mapping to SRL16s
      | for use in pipelining to help achieve timing closure.
      mask init:
      | pipeline_init(gcb,'latency',latency);
      settings: AttributesFormatString=Latency = %<latency>
      mask Display:
      | port_label('input', 1, 'd');
      | port_label('output', 1, 'q');
      | disp(['Z^-', num2str(latency)]);
  pipeline432 : Subsystem  AncestorBlock=casper_library_delays/pipeline  mask(pipeline){latency=2}
      mask help:
      | An explicitly laid-out delay line to avoid mapping to SRL16s
      | for use in pipelining to help achieve timing closure.
      mask init:
      | pipeline_init(gcb,'latency',latency);
      settings: AttributesFormatString=Latency = %<latency>
      mask Display:
      | port_label('input', 1, 'd');
      | port_label('output', 1, 'q');
      | disp(['Z^-', num2str(latency)]);
  pipeline433 : Subsystem  AncestorBlock=casper_library_delays/pipeline  mask(pipeline){latency=2}
      mask help:
      | An explicitly laid-out delay line to avoid mapping to SRL16s
      | for use in pipelining to help achieve timing closure.
      mask init:
      | pipeline_init(gcb,'latency',latency);
      settings: AttributesFormatString=Latency = %<latency>
      mask Display:
      | port_label('input', 1, 'd');
      | port_label('output', 1, 'q');
      | disp(['Z^-', num2str(latency)]);
  pipeline434 : Subsystem  AncestorBlock=casper_library_delays/pipeline  mask(pipeline){latency=2}
      mask help:
      | An explicitly laid-out delay line to avoid mapping to SRL16s
      | for use in pipelining to help achieve timing closure.
      mask init:
      | pipeline_init(gcb,'latency',latency);
      settings: AttributesFormatString=Latency = %<latency>
      mask Display:
      | port_label('input', 1, 'd');
      | port_label('output', 1, 'q');
      | disp(['Z^-', num2str(latency)]);
  pipeline435 : Subsystem  AncestorBlock=casper_library_delays/pipeline  mask(pipeline){latency=3}
      mask help:
      | An explicitly laid-out delay line to avoid mapping to SRL16s
      | for use in pipelining to help achieve timing closure.
      mask init:
      | pipeline_init(gcb,'latency',latency);
      settings: AttributesFormatString=Latency = %<latency>
      mask Display:
      | port_label('input', 1, 'd');
      | port_label('output', 1, 'q');
      | disp(['Z^-', num2str(latency)]);
  pipeline436 : Subsystem  AncestorBlock=casper_library_delays/pipeline  mask(pipeline){latency=3}
      mask help:
      | An explicitly laid-out delay line to avoid mapping to SRL16s
      | for use in pipelining to help achieve timing closure.
      mask init:
      | pipeline_init(gcb,'latency',latency);
      settings: AttributesFormatString=Latency = %<latency>
      mask Display:
      | port_label('input', 1, 'd');
      | port_label('output', 1, 'q');
      | disp(['Z^-', num2str(latency)]);
  pipeline437 : Subsystem  AncestorBlock=casper_library_delays/pipeline  mask(pipeline){latency=3}
      mask help:
      | An explicitly laid-out delay line to avoid mapping to SRL16s
      | for use in pipelining to help achieve timing closure.
      mask init:
      | pipeline_init(gcb,'latency',latency);
      settings: AttributesFormatString=Latency = %<latency>
      mask Display:
      | port_label('input', 1, 'd');
      | port_label('output', 1, 'q');
      | disp(['Z^-', num2str(latency)]);
  pipeline438 : Subsystem  AncestorBlock=casper_library_delays/pipeline  mask(pipeline){latency=3}
      mask help:
      | An explicitly laid-out delay line to avoid mapping to SRL16s
      | for use in pipelining to help achieve timing closure.
      mask init:
      | pipeline_init(gcb,'latency',latency);
      settings: AttributesFormatString=Latency = %<latency>
      mask Display:
      | port_label('input', 1, 'd');
      | port_label('output', 1, 'q');
      | disp(['Z^-', num2str(latency)]);
  pipeline439 : Subsystem  AncestorBlock=casper_library_delays/pipeline  mask(pipeline){latency=2}
      mask help:
      | An explicitly laid-out delay line to avoid mapping to SRL16s
      | for use in pipelining to help achieve timing closure.
      mask init:
      | pipeline_init(gcb,'latency',latency);
      settings: AttributesFormatString=Latency = %<latency>
      mask Display:
      | port_label('input', 1, 'd');
      | port_label('output', 1, 'q');
      | disp(['Z^-', num2str(latency)]);
  pipeline440 : Subsystem  AncestorBlock=casper_library_delays/pipeline  mask(pipeline){latency=2}
      mask help:
      | An explicitly laid-out delay line to avoid mapping to SRL16s
      | for use in pipelining to help achieve timing closure.
      mask init:
      | pipeline_init(gcb,'latency',latency);
      settings: AttributesFormatString=Latency = %<latency>
      mask Display:
      | port_label('input', 1, 'd');
      | port_label('output', 1, 'q');
      | disp(['Z^-', num2str(latency)]);
  pipeline441 : Subsystem  AncestorBlock=casper_library_delays/pipeline  mask(pipeline){latency=2}
      mask help:
      | An explicitly laid-out delay line to avoid mapping to SRL16s
      | for use in pipelining to help achieve timing closure.
      mask init:
      | pipeline_init(gcb,'latency',latency);
      settings: AttributesFormatString=Latency = %<latency>
      mask Display:
      | port_label('input', 1, 'd');
      | port_label('output', 1, 'q');
      | disp(['Z^-', num2str(latency)]);
  pipeline442 : Subsystem  AncestorBlock=casper_library_delays/pipeline  mask(pipeline){latency=2}
      mask help:
      | An explicitly laid-out delay line to avoid mapping to SRL16s
      | for use in pipelining to help achieve timing closure.
      mask init:
      | pipeline_init(gcb,'latency',latency);
      settings: AttributesFormatString=Latency = %<latency>
      mask Display:
      | port_label('input', 1, 'd');
      | port_label('output', 1, 'q');
      | disp(['Z^-', num2str(latency)]);
  pipeline445 : Subsystem  AncestorBlock=casper_library_delays/pipeline  mask(pipeline){latency=2}
      mask help:
      | An explicitly laid-out delay line to avoid mapping to SRL16s
      | for use in pipelining to help achieve timing closure.
      mask init:
      | pipeline_init(gcb,'latency',latency);
      settings: AttributesFormatString=Latency = %<latency>
      mask Display:
      | port_label('input', 1, 'd');
      | port_label('output', 1, 'q');
      | disp(['Z^-', num2str(latency)]);
  pipeline446 : Subsystem  AncestorBlock=casper_library_delays/pipeline  mask(pipeline){latency=2}
      mask help:
      | An explicitly laid-out delay line to avoid mapping to SRL16s
      | for use in pipelining to help achieve timing closure.
      mask init:
      | pipeline_init(gcb,'latency',latency);
      settings: AttributesFormatString=Latency = %<latency>
      mask Display:
      | port_label('input', 1, 'd');
      | port_label('output', 1, 'q');
      | disp(['Z^-', num2str(latency)]);
  pipeline447 : Subsystem  AncestorBlock=casper_library_delays/pipeline  mask(pipeline){latency=2}
      mask help:
      | An explicitly laid-out delay line to avoid mapping to SRL16s
      | for use in pipelining to help achieve timing closure.
      mask init:
      | pipeline_init(gcb,'latency',latency);
      settings: AttributesFormatString=Latency = %<latency>
      mask Display:
      | port_label('input', 1, 'd');
      | port_label('output', 1, 'q');
      | disp(['Z^-', num2str(latency)]);
  pipeline448 : Subsystem  AncestorBlock=casper_library_delays/pipeline  mask(pipeline){latency=2}
      mask help:
      | An explicitly laid-out delay line to avoid mapping to SRL16s
      | for use in pipelining to help achieve timing closure.
      mask init:
      | pipeline_init(gcb,'latency',latency);
      settings: AttributesFormatString=Latency = %<latency>
      mask Display:
      | port_label('input', 1, 'd');
      | port_label('output', 1, 'q');
      | disp(['Z^-', num2str(latency)]);
  pipeline449 : Subsystem  AncestorBlock=casper_library_delays/pipeline  mask(pipeline){latency=2}
      mask help:
      | An explicitly laid-out delay line to avoid mapping to SRL16s
      | for use in pipelining to help achieve timing closure.
      mask init:
      | pipeline_init(gcb,'latency',latency);
      settings: AttributesFormatString=Latency = %<latency>
      mask Display:
      | port_label('input', 1, 'd');
      | port_label('output', 1, 'q');
      | disp(['Z^-', num2str(latency)]);
  pipeline450 : Subsystem  AncestorBlock=casper_library_delays/pipeline  mask(pipeline){latency=1}
      mask help:
      | An explicitly laid-out delay line to avoid mapping to SRL16s
      | for use in pipelining to help achieve timing closure.
      mask init:
      | pipeline_init(gcb,'latency',latency);
      settings: AttributesFormatString=Latency = %<latency>
      mask Display:
      | port_label('input', 1, 'd');
      | port_label('output', 1, 'q');
      | disp(['Z^-', num2str(latency)]);
  pipeline451 : Subsystem  AncestorBlock=casper_library_delays/pipeline  mask(pipeline){latency=1}
      mask help:
      | An explicitly laid-out delay line to avoid mapping to SRL16s
      | for use in pipelining to help achieve timing closure.
      mask init:
      | pipeline_init(gcb,'latency',latency);
      settings: AttributesFormatString=Latency = %<latency>
      mask Display:
      | port_label('input', 1, 'd');
      | port_label('output', 1, 'q');
      | disp(['Z^-', num2str(latency)]);
  pipeline452 : Subsystem  AncestorBlock=casper_library_delays/pipeline  mask(pipeline){latency=1}
      mask help:
      | An explicitly laid-out delay line to avoid mapping to SRL16s
      | for use in pipelining to help achieve timing closure.
      mask init:
      | pipeline_init(gcb,'latency',latency);
      settings: AttributesFormatString=Latency = %<latency>
      mask Display:
      | port_label('input', 1, 'd');
      | port_label('output', 1, 'q');
      | disp(['Z^-', num2str(latency)]);
  pipeline453 : Subsystem  AncestorBlock=casper_library_delays/pipeline  mask(pipeline){latency=3}
      mask help:
      | An explicitly laid-out delay line to avoid mapping to SRL16s
      | for use in pipelining to help achieve timing closure.
      mask init:
      | pipeline_init(gcb,'latency',latency);
      settings: AttributesFormatString=Latency = %<latency>
      mask Display:
      | port_label('input', 1, 'd');
      | port_label('output', 1, 'q');
      | disp(['Z^-', num2str(latency)]);
  pipeline457 : Subsystem  AncestorBlock=casper_library_delays/pipeline  mask(pipeline){latency=2}
      mask help:
      | An explicitly laid-out delay line to avoid mapping to SRL16s
      | for use in pipelining to help achieve timing closure.
      mask init:
      | pipeline_init(gcb,'latency',latency);
      settings: AttributesFormatString=Latency = %<latency>
      mask Display:
      | port_label('input', 1, 'd');
      | port_label('output', 1, 'q');
      | disp(['Z^-', num2str(latency)]);
  pipeline458 : Subsystem  AncestorBlock=casper_library_delays/pipeline  mask(pipeline){latency=2}
      mask help:
      | An explicitly laid-out delay line to avoid mapping to SRL16s
      | for use in pipelining to help achieve timing closure.
      mask init:
      | pipeline_init(gcb,'latency',latency);
      settings: AttributesFormatString=Latency = %<latency>
      mask Display:
      | port_label('input', 1, 'd');
      | port_label('output', 1, 'q');
      | disp(['Z^-', num2str(latency)]);
  pipeline461 : Subsystem  AncestorBlock=casper_library_delays/pipeline  mask(pipeline){latency=2}
      mask help:
      | An explicitly laid-out delay line to avoid mapping to SRL16s
      | for use in pipelining to help achieve timing closure.
      mask init:
      | pipeline_init(gcb,'latency',latency);
      settings: AttributesFormatString=Latency = %<latency>
      mask Display:
      | port_label('input', 1, 'd');
      | port_label('output', 1, 'q');
      | disp(['Z^-', num2str(latency)]);
  pipeline5 : Subsystem  AncestorBlock=casper_library_delays/pipeline  mask(pipeline){latency=2}
      mask help:
      | An explicitly laid-out delay line to avoid mapping to SRL16s
      | for use in pipelining to help achieve timing closure.
      mask init:
      | pipeline_init(gcb,'latency',latency);
      settings: AttributesFormatString=Latency = %<latency>
      mask Display:
      | port_label('input', 1, 'd');
      | port_label('output', 1, 'q');
      | disp(['Z^-', num2str(latency)]);
  pipeline52 : Subsystem  AncestorBlock=casper_library_delays/pipeline  mask(pipeline){latency=2}
      mask help:
      | An explicitly laid-out delay line to avoid mapping to SRL16s
      | for use in pipelining to help achieve timing closure.
      mask init:
      | pipeline_init(gcb,'latency',latency);
      settings: AttributesFormatString=Latency = %<latency>
      mask Display:
      | port_label('input', 1, 'd');
      | port_label('output', 1, 'q');
      | disp(['Z^-', num2str(latency)]);
  pipeline59 : Subsystem  AncestorBlock=casper_library_delays/pipeline  mask(pipeline){latency=2}
      mask help:
      | An explicitly laid-out delay line to avoid mapping to SRL16s
      | for use in pipelining to help achieve timing closure.
      mask init:
      | pipeline_init(gcb,'latency',latency);
      settings: AttributesFormatString=Latency = %<latency>
      mask Display:
      | port_label('input', 1, 'd');
      | port_label('output', 1, 'q');
      | disp(['Z^-', num2str(latency)]);
  pipeline6 : Subsystem  AncestorBlock=casper_library_delays/pipeline  mask(pipeline){latency=2}
      mask help:
      | An explicitly laid-out delay line to avoid mapping to SRL16s
      | for use in pipelining to help achieve timing closure.
      mask init:
      | pipeline_init(gcb,'latency',latency);
      settings: AttributesFormatString=Latency = %<latency>
      mask Display:
      | port_label('input', 1, 'd');
      | port_label('output', 1, 'q');
      | disp(['Z^-', num2str(latency)]);
  pipeline66 : Subsystem  AncestorBlock=casper_library_delays/pipeline  mask(pipeline){latency=2}
      mask help:
      | An explicitly laid-out delay line to avoid mapping to SRL16s
      | for use in pipelining to help achieve timing closure.
      mask init:
      | pipeline_init(gcb,'latency',latency);
      settings: AttributesFormatString=Latency = %<latency>
      mask Display:
      | port_label('input', 1, 'd');
      | port_label('output', 1, 'q');
      | disp(['Z^-', num2str(latency)]);
  pipeline7 : Subsystem  AncestorBlock=casper_library_delays/pipeline  mask(pipeline){latency=2}
      mask help:
      | An explicitly laid-out delay line to avoid mapping to SRL16s
      | for use in pipelining to help achieve timing closure.
      mask init:
      | pipeline_init(gcb,'latency',latency);
      settings: AttributesFormatString=Latency = %<latency>
      mask Display:
      | port_label('input', 1, 'd');
      | port_label('output', 1, 'q');
      | disp(['Z^-', num2str(latency)]);
  pipeline9 : Subsystem  AncestorBlock=casper_library_delays/pipeline  mask(pipeline){latency=2}
      mask help:
      | An explicitly laid-out delay line to avoid mapping to SRL16s
      | for use in pipelining to help achieve timing closure.
      mask init:
      | pipeline_init(gcb,'latency',latency);
      settings: AttributesFormatString=Latency = %<latency>
      mask Display:
      | port_label('input', 1, 'd');
      | port_label('output', 1, 'q');
      | disp(['Z^-', num2str(latency)]);
  pipeline93 : Subsystem  AncestorBlock=casper_library_delays/pipeline  mask(pipeline){latency=2}
      mask help:
      | An explicitly laid-out delay line to avoid mapping to SRL16s
      | for use in pipelining to help achieve timing closure.
      mask init:
      | pipeline_init(gcb,'latency',latency);
      settings: AttributesFormatString=Latency = %<latency>
      mask Display:
      | port_label('input', 1, 'd');
      | port_label('output', 1, 'q');
      | disp(['Z^-', num2str(latency)]);
  pol0_num_pkts : Subsystem  Tag=xps:sw_reg  AncestorBlock=xps_library/software_register  mask(swreg){io_dir=From Processor, io_delay=1, sample_period=1, names=pol0_num_pkts, bitwidths=32, bin_pts=0, arith_types=0, sim_port=on, show_format=on}
      mask prompts: io_dir "I/O direction"; io_delay "I/O delay"; sample_period "Sample period"; names "Bitfield names [msb...lsb]"; bitwidths "Bitfield widths"; bin_pts "Bitfield binary pts"; arith_types "Bitfield types, ufix=0, fix=1, bool=2"; sim_port "Provide sim input/output?"; show_format "Print format string?"
      mask help: A 32-bit software-accessible register. Can be divided into bitfields of varying widths and types using the fields in the block mask.
      mask init:
      | swreg_init(gcb)
      settings: AttributesFormatString=1input:uf32.0 = 32 bits
      mask TypeOptions io_dir: To Processor | From Processor
      mask Callback io_dir:
      | mask_enables = get_param(gcb, 'MaskEnables');
      | mask_names = get_param(gcb, 'MaskNames');
      | if strcmp(get_param(gcb, 'io_dir'), 'To Processor'),
      |     mask_enables{ismember(mask_names, 'sample_period')} = 'off';
      | else
      |     mask_enables{ismember(mask_names, 'sample_period')} = 'on';
      | end
      | set_param(gcb, 'MaskEnables', mask_enables);
  pol0_sample_offset : Subsystem  Tag=xps:sw_reg  AncestorBlock=xps_library/software_register  mask(swreg){io_dir=From Processor, io_delay=1, sample_period=1, names=pol0_sample_offset, bitwidths=18, bin_pts=0, arith_types=0, sim_port=on, show_format=on}
      mask prompts: io_dir "I/O direction"; io_delay "I/O delay"; sample_period "Sample period"; names "Bitfield names [msb...lsb]"; bitwidths "Bitfield widths"; bin_pts "Bitfield binary pts"; arith_types "Bitfield types, ufix=0, fix=1, bool=2"; sim_port "Provide sim input/output?"; show_format "Print format string?"
      mask help: A 32-bit software-accessible register. Can be divided into bitfields of varying widths and types using the fields in the block mask.
      mask init:
      | swreg_init(gcb)
      settings: AttributesFormatString=1input:uf18.0 = 18 bits
      mask TypeOptions io_dir: To Processor | From Processor
      mask Callback io_dir:
      | mask_enables = get_param(gcb, 'MaskEnables');
      | mask_names = get_param(gcb, 'MaskNames');
      | if strcmp(get_param(gcb, 'io_dir'), 'To Processor'),
      |     mask_enables{ismember(mask_names, 'sample_period')} = 'off';
      | else
      |     mask_enables{ismember(mask_names, 'sample_period')} = 'on';
      | end
      | set_param(gcb, 'MaskEnables', mask_enables);
  pol1_num_pkts : Subsystem  Tag=xps:sw_reg  AncestorBlock=xps_library/software_register  mask(swreg){io_dir=From Processor, io_delay=1, sample_period=1, names=pol1_num_pkts, bitwidths=32, bin_pts=0, arith_types=0, sim_port=on, show_format=on}
      mask prompts: io_dir "I/O direction"; io_delay "I/O delay"; sample_period "Sample period"; names "Bitfield names [msb...lsb]"; bitwidths "Bitfield widths"; bin_pts "Bitfield binary pts"; arith_types "Bitfield types, ufix=0, fix=1, bool=2"; sim_port "Provide sim input/output?"; show_format "Print format string?"
      mask help: A 32-bit software-accessible register. Can be divided into bitfields of varying widths and types using the fields in the block mask.
      mask init:
      | swreg_init(gcb)
      settings: AttributesFormatString=1input:uf32.0 = 32 bits
      mask TypeOptions io_dir: To Processor | From Processor
      mask Callback io_dir:
      | mask_enables = get_param(gcb, 'MaskEnables');
      | mask_names = get_param(gcb, 'MaskNames');
      | if strcmp(get_param(gcb, 'io_dir'), 'To Processor'),
      |     mask_enables{ismember(mask_names, 'sample_period')} = 'off';
      | else
      |     mask_enables{ismember(mask_names, 'sample_period')} = 'on';
      | end
      | set_param(gcb, 'MaskEnables', mask_enables);
  pol1_sample_offset : Subsystem  Tag=xps:sw_reg  AncestorBlock=xps_library/software_register  mask(swreg){io_dir=From Processor, io_delay=1, sample_period=1, names=pol1_sample_offset, bitwidths=18, bin_pts=0, arith_types=0, sim_port=on, show_format=on}
      mask prompts: io_dir "I/O direction"; io_delay "I/O delay"; sample_period "Sample period"; names "Bitfield names [msb...lsb]"; bitwidths "Bitfield widths"; bin_pts "Bitfield binary pts"; arith_types "Bitfield types, ufix=0, fix=1, bool=2"; sim_port "Provide sim input/output?"; show_format "Print format string?"
      mask help: A 32-bit software-accessible register. Can be divided into bitfields of varying widths and types using the fields in the block mask.
      mask init:
      | swreg_init(gcb)
      settings: AttributesFormatString=1input:uf18.0 = 18 bits
      mask TypeOptions io_dir: To Processor | From Processor
      mask Callback io_dir:
      | mask_enables = get_param(gcb, 'MaskEnables');
      | mask_names = get_param(gcb, 'MaskNames');
      | if strcmp(get_param(gcb, 'io_dir'), 'To Processor'),
      |     mask_enables{ismember(mask_names, 'sample_period')} = 'off';
      | else
      |     mask_enables{ismember(mask_names, 'sample_period')} = 'on';
      | end
      | set_param(gcb, 'MaskEnables', mask_enables);
  pol_traffic_trigger : Subsystem  Tag=xps:sw_reg  AncestorBlock=xps_library/software_register  mask(swreg){io_dir=From Processor, io_delay=1, sample_period=1, names=[pol0_tx_trigger pol1_tx_trigger], bitwidths=[1 1], bin_pts=[0 0], arith_types=[2 2], sim_port=on, show_format=on}
      mask prompts: io_dir "I/O direction"; io_delay "I/O delay"; sample_period "Sample period"; names "Bitfield names [msb...lsb]"; bitwidths "Bitfield widths"; bin_pts "Bitfield binary pts"; arith_types "Bitfield types, ufix=0, fix=1, bool=2"; sim_port "Provide sim input/output?"; show_format "Print format string?"
      mask help: A 32-bit software-accessible register. Can be divided into bitfields of varying widths and types using the fields in the block mask.
      mask init:
      | swreg_init(gcb)
      settings: AttributesFormatString=2 inputs:b,b = 2 bits
      mask TypeOptions io_dir: To Processor | From Processor
      mask Callback io_dir:
      | mask_enables = get_param(gcb, 'MaskEnables');
      | mask_names = get_param(gcb, 'MaskNames');
      | if strcmp(get_param(gcb, 'io_dir'), 'To Processor'),
      |     mask_enables{ismember(mask_names, 'sample_period')} = 'off';
      | else
      |     mask_enables{ismember(mask_names, 'sample_period')} = 'on';
      | end
      | set_param(gcb, 'MaskEnables', mask_enables);
  pol_tx_always_on : Subsystem  Tag=xps:sw_reg  AncestorBlock=xps_library/software_register  mask(swreg){io_dir=From Processor, io_delay=1, sample_period=1, names=[pol0_tx_always_on pol1_tx_always_on], bitwidths=[1 1], bin_pts=[0 0], arith_types=[2 2], sim_port=on, show_format=on}
      mask prompts: io_dir "I/O direction"; io_delay "I/O delay"; sample_period "Sample period"; names "Bitfield names [msb...lsb]"; bitwidths "Bitfield widths"; bin_pts "Bitfield binary pts"; arith_types "Bitfield types, ufix=0, fix=1, bool=2"; sim_port "Provide sim input/output?"; show_format "Print format string?"
      mask help: A 32-bit software-accessible register. Can be divided into bitfields of varying widths and types using the fields in the block mask.
      mask init:
      | swreg_init(gcb)
      settings: AttributesFormatString=2 inputs:b,b = 2 bits
      mask TypeOptions io_dir: To Processor | From Processor
      mask Callback io_dir:
      | mask_enables = get_param(gcb, 'MaskEnables');
      | mask_names = get_param(gcb, 'MaskNames');
      | if strcmp(get_param(gcb, 'io_dir'), 'To Processor'),
      |     mask_enables{ismember(mask_names, 'sample_period')} = 'off';
      | else
      |     mask_enables{ismember(mask_names, 'sample_period')} = 'on';
      | end
      | set_param(gcb, 'MaskEnables', mask_enables);
  ramp{0..3} (4 alike) : xbsIndex_r4/Counter  cnt_type=Free Running  cnt_to=Inf  operation=Up  start_count=0  cnt_by_val=1  arith_type=Unsigned  n_bits=64  bin_pt=0  load_pin=off  rst=on  en=on  explicit_period=on  period=1  use_behavioral_HDL=off  implementation=Fabric  dbl_ovrd=off  block_type=counter
  ramp80 : xbsIndex_r4/Counter  cnt_type=Free Running  cnt_to=Inf  operation=Up  start_count=0  cnt_by_val=1  arith_type=Unsigned  n_bits=79  bin_pt=0  load_pin=off  rst=on  en=off  explicit_period=on  period=1  use_behavioral_HDL=off  implementation=Fabric  dbl_ovrd=off  block_type=counter
  rd_addr{0..3} (4 alike) : xbsIndex_r4/Counter  cnt_type=Free Running  cnt_to=Inf  operation=Up  start_count=0  cnt_by_val=1  arith_type=Unsigned  n_bits=8  bin_pt=0  load_pin=off  rst=on  en=on  explicit_period=on  period=1  use_behavioral_HDL=off  implementation=Fabric  dbl_ovrd=off  block_type=counter
  rd_arm{,1..3} (4 alike) : xbsIndex_r4/Register  init=0  rst=on  en=on  dbl_ovrd=off  block_type=register
  receptor_id : Subsystem  Tag=xps:sw_reg  AncestorBlock=xps_library/software_register  mask(swreg){io_dir=From Processor, io_delay=1, sample_period=1, names=[receptor_id pol0_id pol1_id], bitwidths=[14 2 2], bin_pts=[0 0 0], arith_types=[0 0 0], sim_port=on, show_format=on}
      mask prompts: io_dir "I/O direction"; io_delay "I/O delay"; sample_period "Sample period"; names "Bitfield names [msb...lsb]"; bitwidths "Bitfield widths"; bin_pts "Bitfield binary pts"; arith_types "Bitfield types, ufix=0, fix=1, bool=2"; sim_port "Provide sim input/output?"; show_format "Print format string?"
      mask help: A 32-bit software-accessible register. Can be divided into bitfields of varying widths and types using the fields in the block mask.
      mask init:
      | swreg_init(gcb)
      settings: AttributesFormatString=3 inputs:uf14.0,uf2.0,uf2.0 = 18 bits
      mask TypeOptions io_dir: To Processor | From Processor
      mask Callback io_dir:
      | mask_enables = get_param(gcb, 'MaskEnables');
      | mask_names = get_param(gcb, 'MaskNames');
      | if strcmp(get_param(gcb, 'io_dir'), 'To Processor'),
      |     mask_enables{ismember(mask_names, 'sample_period')} = 'off';
      | else
      |     mask_enables{ismember(mask_names, 'sample_period')} = 'on';
      | end
      | set_param(gcb, 'MaskEnables', mask_enables);
  rpt_en_cwg0 : Subsystem  Tag=xps:sw_reg  AncestorBlock=xps_library/software_register  mask(swreg){io_dir=From Processor, io_delay=1, sample_period=1, names=[en dummy], bitwidths=[1 31], bin_pts=[0 0], arith_types=[0 0], sim_port=on, show_format=on}
      mask prompts: io_dir "I/O direction"; io_delay "I/O delay"; sample_period "Sample period"; names "Bitfield names [msb...lsb]"; bitwidths "Bitfield widths"; bin_pts "Bitfield binary pts"; arith_types "Bitfield types, ufix=0, fix=1, bool=2"; sim_port "Provide sim input/output?"; show_format "Print format string?"
      mask help: A 32-bit software-accessible register. Can be divided into bitfields of varying widths and types using the fields in the block mask.
      mask init:
      | swreg_init(gcb)
      settings: AttributesFormatString=2 inputs:uf1.0,uf31.0 = 32 bits
      mask TypeOptions io_dir: To Processor | From Processor
      mask Callback io_dir:
      | mask_enables = get_param(gcb, 'MaskEnables');
      | mask_names = get_param(gcb, 'MaskNames');
      | if strcmp(get_param(gcb, 'io_dir'), 'To Processor'),
      |     mask_enables{ismember(mask_names, 'sample_period')} = 'off';
      | else
      |     mask_enables{ismember(mask_names, 'sample_period')} = 'on';
      | end
      | set_param(gcb, 'MaskEnables', mask_enables);
  rpt_length_cwg0 : Subsystem  Tag=xps:sw_reg  AncestorBlock=xps_library/software_register  mask(swreg){io_dir=From Processor, io_delay=1, sample_period=1, names=cwg0_repeat_length, bitwidths=32, bin_pts=0, arith_types=0, sim_port=on, show_format=on}
      mask prompts: io_dir "I/O direction"; io_delay "I/O delay"; sample_period "Sample period"; names "Bitfield names [msb...lsb]"; bitwidths "Bitfield widths"; bin_pts "Bitfield binary pts"; arith_types "Bitfield types, ufix=0, fix=1, bool=2"; sim_port "Provide sim input/output?"; show_format "Print format string?"
      mask help: A 32-bit software-accessible register. Can be divided into bitfields of varying widths and types using the fields in the block mask.
      mask init:
      | swreg_init(gcb)
      settings: AttributesFormatString=1input:uf32.0 = 32 bits
      mask TypeOptions io_dir: To Processor | From Processor
      mask Callback io_dir:
      | mask_enables = get_param(gcb, 'MaskEnables');
      | mask_names = get_param(gcb, 'MaskNames');
      | if strcmp(get_param(gcb, 'io_dir'), 'To Processor'),
      |     mask_enables{ismember(mask_names, 'sample_period')} = 'off';
      | else
      |     mask_enables{ismember(mask_names, 'sample_period')} = 'on';
      | end
      | set_param(gcb, 'MaskEnables', mask_enables);
  sample_masking : Subsystem  mask{dbwidth=1}
      mask prompts: dbwidth "Data bitwidth:"
  scale_cwg0 : Subsystem  Tag=xps:sw_reg  AncestorBlock=xps_library/software_register  mask(swreg){io_dir=From Processor, io_delay=1, sample_period=1, names=[scale dummy], bitwidths=16, bin_pts=15, arith_types=0, sim_port=on, show_format=on}
      mask prompts: io_dir "I/O direction"; io_delay "I/O delay"; sample_period "Sample period"; names "Bitfield names [msb...lsb]"; bitwidths "Bitfield widths"; bin_pts "Bitfield binary pts"; arith_types "Bitfield types, ufix=0, fix=1, bool=2"; sim_port "Provide sim input/output?"; show_format "Print format string?"
      mask help: A 32-bit software-accessible register. Can be divided into bitfields of varying widths and types using the fields in the block mask.
      mask init:
      | swreg_init(gcb)
      settings: AttributesFormatString=2 inputs:uf16.15,uf16.15 = 32 bits
      mask TypeOptions io_dir: To Processor | From Processor
      mask Callback io_dir:
      | mask_enables = get_param(gcb, 'MaskEnables');
      | mask_names = get_param(gcb, 'MaskNames');
      | if strcmp(get_param(gcb, 'io_dir'), 'To Processor'),
      |     mask_enables{ismember(mask_names, 'sample_period')} = 'off';
      | else
      |     mask_enables{ismember(mask_names, 'sample_period')} = 'on';
      | end
      | set_param(gcb, 'MaskEnables', mask_enables);
  scale_out0 : Subsystem  Tag=xps:sw_reg  AncestorBlock=xps_library/software_register  mask(swreg){io_dir=From Processor, io_delay=1, sample_period=1, names=[scale dummy], bitwidths=16, bin_pts=15, arith_types=0, sim_port=on, show_format=on}
      mask prompts: io_dir "I/O direction"; io_delay "I/O delay"; sample_period "Sample period"; names "Bitfield names [msb...lsb]"; bitwidths "Bitfield widths"; bin_pts "Bitfield binary pts"; arith_types "Bitfield types, ufix=0, fix=1, bool=2"; sim_port "Provide sim input/output?"; show_format "Print format string?"
      mask help: A 32-bit software-accessible register. Can be divided into bitfields of varying widths and types using the fields in the block mask.
      mask init:
      | swreg_init(gcb)
      settings: AttributesFormatString=2 inputs:uf16.15,uf16.15 = 32 bits
      mask TypeOptions io_dir: To Processor | From Processor
      mask Callback io_dir:
      | mask_enables = get_param(gcb, 'MaskEnables');
      | mask_names = get_param(gcb, 'MaskNames');
      | if strcmp(get_param(gcb, 'io_dir'), 'To Processor'),
      |     mask_enables{ismember(mask_names, 'sample_period')} = 'off';
      | else
      |     mask_enables{ismember(mask_names, 'sample_period')} = 'on';
      | end
      | set_param(gcb, 'MaskEnables', mask_enables);
  slice1 : xbsIndex_r4/Slice  nbits=32  boolean_output=off  mode=Lower Bit Location + Width  bit1=-7  base1=MSB of Input  bit0=0  base0=LSB of Input  dbl_ovrd=off  block_type=slice
  slice2 : xbsIndex_r4/Slice  nbits=32  boolean_output=off  mode=Lower Bit Location + Width  bit1=-32  base1=MSB of Input  bit0=32  base0=LSB of Input  dbl_ovrd=off  block_type=slice
  spead_pack4 : Subsystem  Tag=casper:spead_pack  AncestorBlock=casper_library_communications/spead_pack  mask(pkt_pack_mask){max_pkt_len_bits=10, header_ids=0x1600, 0x3101, 0x3102, header_ind_ids=0x3300, spead_msw=64, spead_lsw=48, spead_version=4, bytes_per_word=8}
      mask prompts: max_pkt_len_bits "Max pkt length, 2^? 64-bit words"; header_ids "SPEAD direct address IDs (decimal)"; header_ind_ids "SPEAD indirect address IDs (decimal)"; spead_msw "SPEAD Flavour (MSw)"; spead_lsw "SPEAD Flavour (LSw)"; spead_version "SPEAD version"; bytes_per_word "Word size, in bytes"
      mask help:
      | This block generates SPEAD-compliant packets from a datastream.
      |
      | Packets are created with a fixed header followed by a number of 64-bit items.
      |
      | Requires a 64-bit data stream.
      |
      | The data_ready signal is one cycle BEFORE valid data! Does not have to be with a valid signal either.
      mask init:
      | if floor(log2(bytes_per_word)) ~= log2(bytes_per_word)
      |     error('Bytes per word should be a power of two.');
      | end
      | 
      | spead_pack_init(gcb)
  spead_pack5 : Subsystem  Tag=casper:spead_pack  AncestorBlock=casper_library_communications/spead_pack  mask(pkt_pack_mask){max_pkt_len_bits=10, header_ids=0x1600, 0x3101, 0x3102, header_ind_ids=0x3300, spead_msw=64, spead_lsw=48, spead_version=4, bytes_per_word=8}
      mask prompts: max_pkt_len_bits "Max pkt length, 2^? 64-bit words"; header_ids "SPEAD direct address IDs (decimal)"; header_ind_ids "SPEAD indirect address IDs (decimal)"; spead_msw "SPEAD Flavour (MSw)"; spead_lsw "SPEAD Flavour (LSw)"; spead_version "SPEAD version"; bytes_per_word "Word size, in bytes"
      mask help:
      | This block generates SPEAD-compliant packets from a datastream.
      |
      | Packets are created with a fixed header followed by a number of 64-bit items.
      |
      | Requires a 64-bit data stream.
      |
      | The data_ready signal is one cycle BEFORE valid data! Does not have to be with a valid signal either.
      mask init:
      | if floor(log2(bytes_per_word)) ~= log2(bytes_per_word)
      |     error('Bytes per word should be a power of two.');
      | end
      | 
      | spead_pack_init(gcb)
  spead_pack6 : Subsystem  Tag=casper:spead_pack  AncestorBlock=casper_library_communications/spead_pack  mask(pkt_pack_mask){max_pkt_len_bits=10, header_ids=0x1600, 0x3101, 0x3102, header_ind_ids=0x3300, spead_msw=64, spead_lsw=48, spead_version=4, bytes_per_word=8}
      mask prompts: max_pkt_len_bits "Max pkt length, 2^? 64-bit words"; header_ids "SPEAD direct address IDs (decimal)"; header_ind_ids "SPEAD indirect address IDs (decimal)"; spead_msw "SPEAD Flavour (MSw)"; spead_lsw "SPEAD Flavour (LSw)"; spead_version "SPEAD version"; bytes_per_word "Word size, in bytes"
      mask help:
      | This block generates SPEAD-compliant packets from a datastream.
      |
      | Packets are created with a fixed header followed by a number of 64-bit items.
      |
      | Requires a 64-bit data stream.
      |
      | The data_ready signal is one cycle BEFORE valid data! Does not have to be with a valid signal either.
      mask init:
      | if floor(log2(bytes_per_word)) ~= log2(bytes_per_word)
      |     error('Bytes per word should be a power of two.');
      | end
      | 
      | spead_pack_init(gcb)
  spead_pack7 : Subsystem  Tag=casper:spead_pack  AncestorBlock=casper_library_communications/spead_pack  mask(pkt_pack_mask){max_pkt_len_bits=10, header_ids=0x1600, 0x3101, 0x3102, header_ind_ids=0x3300, spead_msw=64, spead_lsw=48, spead_version=4, bytes_per_word=8}
      mask prompts: max_pkt_len_bits "Max pkt length, 2^? 64-bit words"; header_ids "SPEAD direct address IDs (decimal)"; header_ind_ids "SPEAD indirect address IDs (decimal)"; spead_msw "SPEAD Flavour (MSw)"; spead_lsw "SPEAD Flavour (LSw)"; spead_version "SPEAD version"; bytes_per_word "Word size, in bytes"
      mask help:
      | This block generates SPEAD-compliant packets from a datastream.
      |
      | Packets are created with a fixed header followed by a number of 64-bit items.
      |
      | Requires a 64-bit data stream.
      |
      | The data_ready signal is one cycle BEFORE valid data! Does not have to be with a valid signal either.
      mask init:
      | if floor(log2(bytes_per_word)) ~= log2(bytes_per_word)
      |     error('Bytes per word should be a power of two.');
      | end
      | 
      | spead_pack_init(gcb)
  speadsnap_control : Subsystem  Tag=xps:sw_reg  AncestorBlock=xps_library/software_register  mask(swreg){io_dir=From Processor, io_delay=0, sample_period=1, names=[speadsnap_arm], bitwidths=1, bin_pts=0, arith_types=2, sim_port=off, show_format=on}
      mask prompts: io_dir "I/O direction"; io_delay "I/O delay"; sample_period "Sample period"; names "Bitfield names [msb...lsb]"; bitwidths "Bitfield widths"; bin_pts "Bitfield binary pts"; arith_types "Bitfield types, ufix=0, fix=1, bool=2"; sim_port "Provide sim input/output?"; show_format "Print format string?"
      mask help: A 32-bit software-accessible register. Can be divided into bitfields of varying widths and types using the fields in the block mask.
      mask init:
      | swreg_init(gcb)
      settings: AttributesFormatString=1input:b = 1 bits
      mask TypeOptions io_dir: To Processor | From Processor
      mask Callback io_dir:
      | mask_enables = get_param(gcb, 'MaskEnables');
      | mask_names = get_param(gcb, 'MaskNames');
      | if strcmp(get_param(gcb, 'io_dir'), 'To Processor'),
      |     mask_enables{ismember(mask_names, 'sample_period')} = 'off';
      | else
      |     mask_enables{ismember(mask_names, 'sample_period')} = 'on';
      | end
      | set_param(gcb, 'MaskEnables', mask_enables);
  speadtime0_offset : Subsystem  Tag=xps:sw_reg  AncestorBlock=xps_library/software_register  mask(swreg){io_dir=From Processor, io_delay=1, sample_period=1, names=speadtime_offset0, bitwidths=32, bin_pts=0, arith_types=0, sim_port=on, show_format=on}
      mask prompts: io_dir "I/O direction"; io_delay "I/O delay"; sample_period "Sample period"; names "Bitfield names [msb...lsb]"; bitwidths "Bitfield widths"; bin_pts "Bitfield binary pts"; arith_types "Bitfield types, ufix=0, fix=1, bool=2"; sim_port "Provide sim input/output?"; show_format "Print format string?"
      mask help: A 32-bit software-accessible register. Can be divided into bitfields of varying widths and types using the fields in the block mask.
      mask init:
      | swreg_init(gcb)
      settings: AttributesFormatString=1input:uf32.0 = 32 bits
      mask TypeOptions io_dir: To Processor | From Processor
      mask Callback io_dir:
      | mask_enables = get_param(gcb, 'MaskEnables');
      | mask_names = get_param(gcb, 'MaskNames');
      | if strcmp(get_param(gcb, 'io_dir'), 'To Processor'),
      |     mask_enables{ismember(mask_names, 'sample_period')} = 'off';
      | else
      |     mask_enables{ismember(mask_names, 'sample_period')} = 'on';
      | end
      | set_param(gcb, 'MaskEnables', mask_enables);
  speadtime1_offset : Subsystem  Tag=xps:sw_reg  AncestorBlock=xps_library/software_register  mask(swreg){io_dir=From Processor, io_delay=1, sample_period=1, names=speadtime_offset1, bitwidths=32, bin_pts=0, arith_types=0, sim_port=on, show_format=on}
      mask prompts: io_dir "I/O direction"; io_delay "I/O delay"; sample_period "Sample period"; names "Bitfield names [msb...lsb]"; bitwidths "Bitfield widths"; bin_pts "Bitfield binary pts"; arith_types "Bitfield types, ufix=0, fix=1, bool=2"; sim_port "Provide sim input/output?"; show_format "Print format string?"
      mask help: A 32-bit software-accessible register. Can be divided into bitfields of varying widths and types using the fields in the block mask.
      mask init:
      | swreg_init(gcb)
      settings: AttributesFormatString=1input:uf32.0 = 32 bits
      mask TypeOptions io_dir: To Processor | From Processor
      mask Callback io_dir:
      | mask_enables = get_param(gcb, 'MaskEnables');
      | mask_names = get_param(gcb, 'MaskNames');
      | if strcmp(get_param(gcb, 'io_dir'), 'To Processor'),
      |     mask_enables{ismember(mask_names, 'sample_period')} = 'off';
      | else
      |     mask_enables{ismember(mask_names, 'sample_period')} = 'on';
      | end
      | set_param(gcb, 'MaskEnables', mask_enables);
  src_sel_cntrl : Subsystem  Tag=xps:sw_reg  AncestorBlock=xps_library/software_register  mask(swreg){io_dir=From Processor, io_delay=1, sample_period=1, names=[src_sel_0 src_sel_1], bitwidths=[2 2], bin_pts=[0 0], arith_types=[0 0], sim_port=on, show_format=on}
      mask prompts: io_dir "I/O direction"; io_delay "I/O delay"; sample_period "Sample period"; names "Bitfield names [msb...lsb]"; bitwidths "Bitfield widths"; bin_pts "Bitfield binary pts"; arith_types "Bitfield types, ufix=0, fix=1, bool=2"; sim_port "Provide sim input/output?"; show_format "Print format string?"
      mask help: A 32-bit software-accessible register. Can be divided into bitfields of varying widths and types using the fields in the block mask.
      mask init:
      | swreg_init(gcb)
      settings: AttributesFormatString=2 inputs:uf2.0,uf2.0 = 4 bits
      mask TypeOptions io_dir: To Processor | From Processor
      mask Callback io_dir:
      | mask_enables = get_param(gcb, 'MaskEnables');
      | mask_names = get_param(gcb, 'MaskNames');
      | if strcmp(get_param(gcb, 'io_dir'), 'To Processor'),
      |     mask_enables{ismember(mask_names, 'sample_period')} = 'off';
      | else
      |     mask_enables{ismember(mask_names, 'sample_period')} = 'on';
      | end
      | set_param(gcb, 'MaskEnables', mask_enables);
  start_flag_lsw : Subsystem  Tag=xps:sw_reg  AncestorBlock=xps_library/software_register  mask(swreg){io_dir=From Processor, io_delay=1, sample_period=1, names=reg, bitwidths=32, bin_pts=0, arith_types=0, sim_port=on, show_format=on}
      mask prompts: io_dir "I/O direction"; io_delay "I/O delay"; sample_period "Sample period"; names "Bitfield names [msb...lsb]"; bitwidths "Bitfield widths"; bin_pts "Bitfield binary pts"; arith_types "Bitfield types, ufix=0, fix=1, bool=2"; sim_port "Provide sim input/output?"; show_format "Print format string?"
      mask help: A 32-bit software-accessible register. Can be divided into bitfields of varying widths and types using the fields in the block mask.
      mask init:
      | swreg_init(gcb)
      settings: AttributesFormatString=1input:uf32.0 = 32 bits
      mask TypeOptions io_dir: To Processor | From Processor
      mask Callback io_dir:
      | mask_enables = get_param(gcb, 'MaskEnables');
      | mask_names = get_param(gcb, 'MaskNames');
      | if strcmp(get_param(gcb, 'io_dir'), 'To Processor'),
      |     mask_enables{ismember(mask_names, 'sample_period')} = 'off';
      | else
      |     mask_enables{ismember(mask_names, 'sample_period')} = 'on';
      | end
      | set_param(gcb, 'MaskEnables', mask_enables);
  start_flag_msw : Subsystem  Tag=xps:sw_reg  AncestorBlock=xps_library/software_register  mask(swreg){io_dir=From Processor, io_delay=1, sample_period=1, names=reg, bitwidths=32, bin_pts=0, arith_types=0, sim_port=on, show_format=on}
      mask prompts: io_dir "I/O direction"; io_delay "I/O delay"; sample_period "Sample period"; names "Bitfield names [msb...lsb]"; bitwidths "Bitfield widths"; bin_pts "Bitfield binary pts"; arith_types "Bitfield types, ufix=0, fix=1, bool=2"; sim_port "Provide sim input/output?"; show_format "Print format string?"
      mask help: A 32-bit software-accessible register. Can be divided into bitfields of varying widths and types using the fields in the block mask.
      mask init:
      | swreg_init(gcb)
      settings: AttributesFormatString=1input:uf32.0 = 32 bits
      mask TypeOptions io_dir: To Processor | From Processor
      mask Callback io_dir:
      | mask_enables = get_param(gcb, 'MaskEnables');
      | mask_names = get_param(gcb, 'MaskNames');
      | if strcmp(get_param(gcb, 'io_dir'), 'To Processor'),
      |     mask_enables{ismember(mask_names, 'sample_period')} = 'off';
      | else
      |     mask_enables{ismember(mask_names, 'sample_period')} = 'on';
      | end
      | set_param(gcb, 'MaskEnables', mask_enables);
  start_time_lsw : Subsystem  Tag=xps:sw_reg  AncestorBlock=xps_library/software_register  mask(swreg){io_dir=From Processor, io_delay=1, sample_period=1, names=reg, bitwidths=32, bin_pts=0, arith_types=0, sim_port=on, show_format=on}
      mask prompts: io_dir "I/O direction"; io_delay "I/O delay"; sample_period "Sample period"; names "Bitfield names [msb...lsb]"; bitwidths "Bitfield widths"; bin_pts "Bitfield binary pts"; arith_types "Bitfield types, ufix=0, fix=1, bool=2"; sim_port "Provide sim input/output?"; show_format "Print format string?"
      mask help: A 32-bit software-accessible register. Can be divided into bitfields of varying widths and types using the fields in the block mask.
      mask init:
      | swreg_init(gcb)
      settings: AttributesFormatString=1input:uf32.0 = 32 bits
      mask TypeOptions io_dir: To Processor | From Processor
      mask Callback io_dir:
      | mask_enables = get_param(gcb, 'MaskEnables');
      | mask_names = get_param(gcb, 'MaskNames');
      | if strcmp(get_param(gcb, 'io_dir'), 'To Processor'),
      |     mask_enables{ismember(mask_names, 'sample_period')} = 'off';
      | else
      |     mask_enables{ismember(mask_names, 'sample_period')} = 'on';
      | end
      | set_param(gcb, 'MaskEnables', mask_enables);
  start_time_msw : Subsystem  Tag=xps:sw_reg  AncestorBlock=xps_library/software_register  mask(swreg){io_dir=From Processor, io_delay=1, sample_period=1, names=reg, bitwidths=32, bin_pts=0, arith_types=0, sim_port=on, show_format=on}
      mask prompts: io_dir "I/O direction"; io_delay "I/O delay"; sample_period "Sample period"; names "Bitfield names [msb...lsb]"; bitwidths "Bitfield widths"; bin_pts "Bitfield binary pts"; arith_types "Bitfield types, ufix=0, fix=1, bool=2"; sim_port "Provide sim input/output?"; show_format "Print format string?"
      mask help: A 32-bit software-accessible register. Can be divided into bitfields of varying widths and types using the fields in the block mask.
      mask init:
      | swreg_init(gcb)
      settings: AttributesFormatString=1input:uf32.0 = 32 bits
      mask TypeOptions io_dir: To Processor | From Processor
      mask Callback io_dir:
      | mask_enables = get_param(gcb, 'MaskEnables');
      | mask_names = get_param(gcb, 'MaskNames');
      | if strcmp(get_param(gcb, 'io_dir'), 'To Processor'),
      |     mask_enables{ismember(mask_names, 'sample_period')} = 'off';
      | else
      |     mask_enables{ismember(mask_names, 'sample_period')} = 'on';
      | end
      | set_param(gcb, 'MaskEnables', mask_enables);
  sync_gen : Subsystem  mask{zerolsbs=26}
      mask prompts: zerolsbs "No. LSBs to be zero:"
  test_control : Subsystem  Tag=xps:sw_reg  AncestorBlock=xps_library/software_register  mask(swreg){io_dir=From Processor, io_delay=0, sample_period=1, names=[sel_ramp80 rst_ramp80], bitwidths=1, bin_pts=0, arith_types=2, sim_port=on, show_format=on}
      mask prompts: io_dir "I/O direction"; io_delay "I/O delay"; sample_period "Sample period"; names "Bitfield names [msb...lsb]"; bitwidths "Bitfield widths"; bin_pts "Bitfield binary pts"; arith_types "Bitfield types, ufix=0, fix=1, bool=2"; sim_port "Provide sim input/output?"; show_format "Print format string?"
      mask help: A 32-bit software-accessible register. Can be divided into bitfields of varying widths and types using the fields in the block mask.
      mask init:
      | swreg_init(gcb)
      settings: AttributesFormatString=2 inputs:b,b = 2 bits
      mask TypeOptions io_dir: To Processor | From Processor
      mask Callback io_dir:
      | mask_enables = get_param(gcb, 'MaskEnables');
      | mask_names = get_param(gcb, 'MaskNames');
      | if strcmp(get_param(gcb, 'io_dir'), 'To Processor'),
      |     mask_enables{ismember(mask_names, 'sample_period')} = 'off';
      | else
      |     mask_enables{ismember(mask_names, 'sample_period')} = 'on';
      | end
      | set_param(gcb, 'MaskEnables', mask_enables);
  tick_offset_lsw : Subsystem  Tag=xps:sw_reg  AncestorBlock=xps_library/software_register  mask(swreg){io_dir=From Processor, io_delay=1, sample_period=1, names=reg, bitwidths=32, bin_pts=0, arith_types=0, sim_port=on, show_format=on}
      mask prompts: io_dir "I/O direction"; io_delay "I/O delay"; sample_period "Sample period"; names "Bitfield names [msb...lsb]"; bitwidths "Bitfield widths"; bin_pts "Bitfield binary pts"; arith_types "Bitfield types, ufix=0, fix=1, bool=2"; sim_port "Provide sim input/output?"; show_format "Print format string?"
      mask help: A 32-bit software-accessible register. Can be divided into bitfields of varying widths and types using the fields in the block mask.
      mask init:
      | swreg_init(gcb)
      settings: AttributesFormatString=1input:uf32.0 = 32 bits
      mask TypeOptions io_dir: To Processor | From Processor
      mask Callback io_dir:
      | mask_enables = get_param(gcb, 'MaskEnables');
      | mask_names = get_param(gcb, 'MaskNames');
      | if strcmp(get_param(gcb, 'io_dir'), 'To Processor'),
      |     mask_enables{ismember(mask_names, 'sample_period')} = 'off';
      | else
      |     mask_enables{ismember(mask_names, 'sample_period')} = 'on';
      | end
      | set_param(gcb, 'MaskEnables', mask_enables);
  tick_offset_msw : Subsystem  Tag=xps:sw_reg  AncestorBlock=xps_library/software_register  mask(swreg){io_dir=From Processor, io_delay=1, sample_period=1, names=reg, bitwidths=32, bin_pts=0, arith_types=0, sim_port=on, show_format=on}
      mask prompts: io_dir "I/O direction"; io_delay "I/O delay"; sample_period "Sample period"; names "Bitfield names [msb...lsb]"; bitwidths "Bitfield widths"; bin_pts "Bitfield binary pts"; arith_types "Bitfield types, ufix=0, fix=1, bool=2"; sim_port "Provide sim input/output?"; show_format "Print format string?"
      mask help: A 32-bit software-accessible register. Can be divided into bitfields of varying widths and types using the fields in the block mask.
      mask init:
      | swreg_init(gcb)
      settings: AttributesFormatString=1input:uf32.0 = 32 bits
      mask TypeOptions io_dir: To Processor | From Processor
      mask Callback io_dir:
      | mask_enables = get_param(gcb, 'MaskEnables');
      | mask_names = get_param(gcb, 'MaskNames');
      | if strcmp(get_param(gcb, 'io_dir'), 'To Processor'),
      |     mask_enables{ismember(mask_names, 'sample_period')} = 'off';
      | else
      |     mask_enables{ismember(mask_names, 'sample_period')} = 'on';
      | end
      | set_param(gcb, 'MaskEnables', mask_enables);
  ticks_since_mrst : Subsystem
  ts_tvg : Subsystem
  tvg_spead_time_with_pkt_ctr : Subsystem  mask{packetlen_bits=9}
      mask prompts: packetlen_bits "Packet length, num 80-bit words (2^?):"
  unpack_and_reorder : Subsystem
  wr_addr{0..3} (4 alike) : xbsIndex_r4/Counter  cnt_type=Free Running  cnt_to=Inf  operation=Up  start_count=0  cnt_by_val=1  arith_type=Unsigned  n_bits=10  bin_pt=0  load_pin=off  rst=on  en=on  explicit_period=on  period=1  use_behavioral_HDL=off  implementation=Fabric  dbl_ovrd=off  block_type=counter
  tag scope: cnt_rst=global, local_time=global, pfb_bypass=global, ts_tvg_en=global
  wires:
  gbe_porttx/1(in_reg) -> pipeline242/1(d)
  Constant197/1 -> gbe_porttx/1(sim_1)
  Constant75/1 -> gbe_iptx0/1(sim_1)
  Constant77/1 -> gbe_iptx1/1(sim_1)
  Constant78/1 -> gbe_iptx2/1(sim_1)
  Constant79/1 -> gbe_iptx3/1(sim_1)
  Constant80/1 -> digitiser_id/1(sim_1)
  Constant82/1 -> receptor_id/1(sim_1)
  Constant81/1 -> digitiser_id/2(sim_2)
  receptor_id/1(in_receptor_id) -> bus_create1/3(in3)
  Constant165/1 -> receptor_id/2(sim_2)
  Constant84/1 -> receptor_id/3(sim_3)
  [masked_time] -> Delay128/1
  tvg_spead_time_with_pkt_ctr/1(local_time) -> Delay131/1
  tvg_spead_time_with_pkt_ctr/3(tvg_data_pol0) -> Delay133/1
  tvg_spead_time_with_pkt_ctr/4(tvg_data_pol1) -> Delay134/1
  tvg_spead_time_with_pkt_ctr/2(spead_time) -> Delay132/1
  [fifoselect] -> edge_detect37/1(in), Inverter2/1
  Register5/1 -> [speadtime0]  "speadtime0"
  Inverter2/1 -> edge_detect38/1(in)
  edge_detect37/1(out) -> Gateway Out14/1, Register5/2
  edge_detect38/1(out) -> Register6/2
  Register6/1 -> [speadtime1]  "speadtime1"
  [mrst] -> ticks_since_mrst/1(reset)
  [sync] -> ticks_since_mrst/2(sync)
  ticks_since_mrst/1(time64) -> [local_time]  "localtime"
  [msync] -> [sync]  "sync"
  edge_detect20/1(out) -> [mrst]  "mrst"
  edge_detect6/1(out) -> [msync]  "msync"
  edge_detect36/1(out) -> Terminator83/1  "clr_status"
  [local_time] -> slice1/1, slice2/1
  Constant92/1 -> orig_control/3(sim_3)
  Constant149/1 -> orig_control/1(sim_1)
  Constant90/1 -> orig_control/2(sim_2)
  Constant98/1 -> orig_control/6(sim_6)
  Constant95/1 -> orig_control/5(sim_5)
  Constant124/1 -> orig_control/4(sim_4)
  Pulse Generator/1 -> orig_control/8(sim_8)
  [tick_offset] -> ticks_since_mrst/3(offset)
  edge_detect7/1(out) -> [load_tick_offset]  "mrst"
  Constant86/1 -> orig_control/9(sim_9)
  digitiser_id/1(in_digitiser_serial) -> bus_create1/1(in1)
  digitiser_id/2(in_digitiser_type) -> bus_create1/2(in2)
  Constant148/1 -> flag_setup/3(sim_3)
  Constant147/1 -> flag_setup/2(sim_2)
  Constant143/1 -> flag_setup/1(sim_1)
  Counter Free-Running3/1 -> Relational Operator4/2
  Constant152/1 -> Relational Operator4/1
  Relational Operator4/1 -> flag_setup/4(sim_4)
  Constant157/1 -> start_flag_msw/1(sim_1)
  Constant158/1 -> start_flag_lsw/1(sim_1)
  Constant156/1 -> end_flag_msw/1(sim_1)
  Constant155/1 -> end_flag_lsw/1(sim_1)
  Concat18/1 -> Delay83/1  "starttime"
  Concat19/1 -> Delay85/1  "stoptime"
  [flag_start_time] -> Delay80/1
  [local_time] -> Delay79/1, Delay81/1
  [flag_end_time] -> Delay82/1, Delay86/1
  Relational4/1 -> Logical24/2  "start_okay"
  [flag_armed] -> Delay78/1
  Relational5/1 -> Logical42/2  "end_okay"
  Logical24/1 -> Delay55/1  "start_okay"
  Logical42/1 -> Logical35/1  "end_okay"
  edge_detect41/1(out) -> [load_flag_time]  "loadtimes"
  Constant144/1 -> Register1/1
  edge_detect40/1(out) -> [reset_flag_time]  "rst"
  [reset_flag_time] -> Register1/2
  [load_flag_time] -> Register1/3
  Register1/1 -> [flag_armed]  "armed"
  Relational Operator3/1 -> flag_setup/5(sim_5)
  Relational8/1 -> Delay54/1  "zero_stop"
  Constant85/1 -> Relational8/2
  Logical35/1 -> Logical4/2  "eokay"
  Counter Free-Running2/1 -> Relational Operator3/2
  Constant154/1 -> Relational Operator3/1
  Logical43/1 -> sample_masking/2(den_in)
  Constant153/1 -> start_time_msw/1(sim_1)
  Constant159/1 -> start_time_lsw/1(sim_1)
  Constant94/1 -> end_time_msw/1(sim_1)
  Constant76/1 -> end_time_lsw/1(sim_1)
  Relational9/1 -> Logical44/2  "start_okay"
  Relational17/1 -> Logical46/2  "end_okay"
  [start_time] -> Delay72/1
  Relational19/1 -> Delay40/1  "first_sample"
  [end_time] -> Delay75/1
  Relational20/1 -> Delay41/1  "last_sample"
  [sample_end] -> sample_masking/6(sample_end)
  [sample_start] -> sample_masking/5(sample_start)
  sample_masking/2(den_out) -> Delay126/1  "enable"
  sample_masking/3(data_mask) -> Delay127/1  "mask"
  edge_detect11/1(out) -> [reset_en_time]  "reset_en_time"
  Relational Operator5/1 -> control_output/2(sim_2)
  Counter Free-Running4/1 -> Relational Operator6/2, Relational Operator5/2
  Constant142/1 -> Relational Operator5/1
  edge_detect12/1(out) -> [load_en_time]  "load_en_time"
  Concat10/1 -> Delay76/1
  Concat11/1 -> Delay77/1
  Constant88/1 -> Register2/1
  [reset_en_time] -> Register2/2
  [load_en_time] -> Register2/3
  Register2/1 -> [en_armed]  "armed"
  Logical44/1 -> Delay42/1  "start_okay"
  Logical46/1 -> Logical45/1  "end_okay"
  Logical45/1 -> Logical43/2
  Constant99/1 -> Delay70/1
  Relational18/1 -> Delay39/1
  Constant93/1 -> control_output/3(sim_3)
  Constant151/1 -> control_output/4(sim_4)
  Constant96/1 -> Relational Operator6/1
  Relational Operator6/1 -> control_output/1(sim_1)
  [data_enable] -> Delay129/1
  [sample_mask] -> Delay130/1
  Constant150/1 -> tick_offset_msw/1(sim_1)
  Constant176/1 -> tick_offset_lsw/1(sim_1)
  Concat16/1 -> Register3/1
  [load_tick_offset] -> Register3/2
  Register3/1 -> [tick_offset]
  bus_addsub2/1(dout) -> Delay95/1
  bus_addsub4/1(dout) -> bus_convert6/1(din)
  bus_mult/1(a*b) -> [cwg0_tp1], bus_convert/1(din)
  pipeline309/1(q) -> edge_detect12/1(in)
  pipeline320/1(q) -> edge_detect11/1(in)
  pipeline331/1(q) -> [sample_start]
  pipeline339/1(q) -> [sample_end]
  Delay76/1 -> [start_time]
  Delay77/1 -> [end_time]
  Delay83/1 -> [flag_start_time]
  Delay85/1 -> [flag_end_time]
  pipeline206/1(q) -> [gbe_ip3]
  pipeline212/1(q) -> [gbe_ip2]
  pipeline220/1(q) -> [gbe_ip0]
  Delay126/1 -> [data_enable]
  Delay127/1 -> [sample_mask]
  Delay128/1 -> tvg_spead_time_with_pkt_ctr/1(localtime64)
  Delay129/1 -> tvg_spead_time_with_pkt_ctr/2(data_enable)
  Delay130/1 -> tvg_spead_time_with_pkt_ctr/3(data_mask)
  Delay131/1 -> [tvg_ltime]
  Delay132/1 -> [tvg_stime]
  Delay133/1 -> [tvg_pol0]
  Delay134/1 -> [tvg_pol1]
  Delay95/1 -> bus_convert4/1(din)
  Delay139/1 -> bus_addsub4/1(a)
  pipeline350/1(q) -> Concat10/1
  pipeline361/1(q) -> Concat10/2
  pipeline372/1(q) -> Concat11/1
  pipeline383/1(q) -> Concat11/2
  pipeline393/1(q) -> [hdr_0x3101]
  pipeline395/1(q) -> [pol0_id]
  pipeline396/1(q) -> [pol1_id]
  orig_control/1(in_up_cnt_rst) -> pipeline204/1(d)
  pipeline204/1(q) -> edge_detect31/1(in)
  orig_control/2(in_tvg_select0) -> pipeline205/1(d)
  orig_control/3(in_tvg_select1) -> pipeline297/1(d)
  orig_control/4(in_clr_status) -> pipeline394/1(d)
  orig_control/5(in_gbe_rst) -> pipeline405/1(d)
  orig_control/6(in_gbe_txen) -> pipeline416/1(d)
  orig_control/7(in_msync) -> pipeline424/1(d)
  orig_control/8(in_mrst) -> pipeline434/1(d)
  orig_control/9(in_load_tick_offset) -> pipeline445/1(d)
  pipeline445/1(q) -> edge_detect7/1(in)
  pipeline434/1(q) -> edge_detect20/1(in)
  pipeline424/1(q) -> edge_detect6/1(in)
  pipeline405/1(q) -> Terminator82/1
  pipeline394/1(q) -> edge_detect36/1(in)
  pipeline297/1(q) -> [tvg_select1]
  pipeline205/1(q) -> [tvg_select0]
  pipeline213/1(q) -> [gbe_ip1]
  gbe_iptx0/1(in_reg) -> pipeline220/1(d)
  gbe_iptx1/1(in_reg) -> pipeline213/1(d)
  gbe_iptx2/1(in_reg) -> pipeline212/1(d)
  gbe_iptx3/1(in_reg) -> pipeline206/1(d)
  tick_offset_msw/1(in_reg) -> pipeline264/1(d)
  pipeline264/1(q) -> Concat16/1
  tick_offset_lsw/1(in_reg) -> pipeline275/1(d)
  pipeline275/1(q) -> Concat16/2
  slice1/1 -> pipeline298/1(d)
  pipeline298/1(q) -> local_time_lsw1/1(out_reg)
  slice2/1 -> pipeline286/1(d)
  pipeline286/1(q) -> local_time_msw1/1(out_reg)
  end_time_lsw/1(in_reg) -> pipeline383/1(d)
  end_time_msw/1(in_reg) -> pipeline372/1(d)
  start_time_lsw/1(in_reg) -> pipeline361/1(d)
  start_time_msw/1(in_reg) -> pipeline350/1(d)
  control_output/4(in_sample_end) -> pipeline339/1(d)
  control_output/3(in_sample_start) -> pipeline331/1(d)
  control_output/2(in_reset_en_time) -> pipeline320/1(d)
  control_output/1(in_load_en_time) -> pipeline309/1(d)
  bus_create1/1(bus_out) -> pipeline393/1(d)
  receptor_id/2(in_pol0_id) -> pipeline395/1(d)
  receptor_id/3(in_pol1_id) -> pipeline396/1(d)
  flag_setup/1(in_adc_count) -> pipeline397/1(d)
  flag_setup/2(in_adc_flag) -> pipeline398/1(d)
  flag_setup/3(in_ndiode_flag) -> pipeline399/1(d)
  flag_setup/4(in_load_flags) -> pipeline400/1(d)
  flag_setup/5(in_reset_flags) -> pipeline401/1(d)
  pipeline401/1(q) -> edge_detect40/1(in)
  pipeline400/1(q) -> edge_detect41/1(in)
  pipeline399/1(q) -> [ndiode_flag]
  pipeline398/1(q) -> [adc_flag]
  pipeline397/1(q) -> [adc_count]
  start_flag_msw/1(in_reg) -> pipeline402/1(d)
  pipeline402/1(q) -> Concat18/1
  start_flag_lsw/1(in_reg) -> pipeline403/1(d)
  pipeline403/1(q) -> Concat18/2
  end_flag_msw/1(in_reg) -> pipeline404/1(d)
  pipeline404/1(q) -> Concat19/1
  end_flag_lsw/1(in_reg) -> pipeline406/1(d)
  pipeline406/1(q) -> Concat19/2
  pipeline418/1(q) -> bus_mult/2(b)
  pipeline458/1(q) -> bus_addsub2/2(b)
  pipeline461/1(q) -> [cwg_80_1], [cwg_80_0]
  Delay46/1 -> bus_addsub4/2(b)
  Delay38/1 -> Logical46/1, Logical44/1
  Delay39/1 -> Logical45/2
  Delay40/1 -> Delay44/1
  Delay41/1 -> Delay45/1
  Delay42/1 -> Logical43/1
  Delay44/1 -> Delay47/1
  Delay45/1 -> Delay48/1
  Delay47/1 -> sample_masking/3(first_samples)
  Delay48/1 -> sample_masking/4(last_samples)
  Delay54/1 -> Logical35/2
  Delay55/1 -> Logical4/1
  Delay56/1 -> Delay57/1
  Delay57/1 -> Delay58/1
  Delay58/1 -> Delay59/1
  Delay59/1 -> sample_masking/1(timei)
  sample_masking/4(flag_valid) -> Delay60/1
  Delay60/1 -> [flag_en]
  Logical4/1 -> sample_masking/7(flag_en)  "flag_en"
  sample_masking/1(timeo) -> Delay61/1
  Delay61/1 -> [masked_time]
  [local_time] -> Delay63/1
  [en_armed] -> Delay64/1
  [local_time] -> Delay65/1, Delay67/1, Delay71/1, Delay74/1
  [start_time] -> Delay66/1
  [end_time] -> Delay68/1, Delay69/1
  Delay63/1 -> Delay56/1
  Delay64/1 -> Delay38/1
  Delay65/1 -> Relational9/1
  Delay66/1 -> Relational9/2
  Delay67/1 -> Relational17/1
  Delay68/1 -> Relational17/2
  Delay69/1 -> Relational18/1
  Delay70/1 -> Relational18/2
  Delay71/1 -> Relational19/1
  Delay72/1 -> Relational19/2
  Delay74/1 -> Relational20/1
  Delay75/1 -> Relational20/2
  Delay78/1 -> Logical42/1, Logical24/1
  Delay79/1 -> Relational4/1
  Delay80/1 -> Relational4/2
  Delay81/1 -> Relational5/1
  Delay82/1 -> Relational5/2
  Delay86/1 -> Relational8/1
  bus_convert/1(dout) -> [cwg0_tp2], pipeline461/1(d)
  Pulse Generator1/1 -> orig_control/7(sim_7)
  bus_constant1/1(dout) -> Delay139/1
  bus_convert4/1(dout) -> Delay46/1
  bus_convert6/1(dout) -> pipeline417/1(d)
  scale_out0/1(in_scale) -> pipeline418/1(d)
  pipeline217/1(q) -> Slice37/1
  Slice37/1 -> Convert1/1
  Convert1/1 -> [pol0_always_on]
  pipeline222/1(q) -> Slice40/1
  Slice40/1 -> Convert3/1
  Constant174/1 -> pol1_sample_offset/1(sim_1)
  pipeline219/1(q) -> [pol1_offset_data]
  Constant173/1 -> pol0_sample_offset/1(sim_1)
  pipeline218/1(q) -> [pol0_offset_data]
  Constant175/1 -> pol0_num_pkts/1(sim_1)
  pipeline216/1(q) -> [pol0_requested_pkts]
  Constant180/1 -> pol1_num_pkts/1(sim_1)
  pipeline225/1(q) -> [pol1_requested_pkts]
  pipeline227/1(q) -> Slice38/1
  Slice38/1 -> Convert2/1
  Convert2/1 -> [pol1_always_on]
  pipeline416/1(q) -> Terminator64/1
  Delay32/1 -> pol_traffic_trigger/1(sim_1)
  Constant172/1 -> pol_tx_always_on/1(sim_1)
  Constant184/1 -> pol_tx_always_on/2(sim_2)
  pol0_num_pkts/1(in_pol0_num_pkts) -> pipeline216/1(d)
  pol1_num_pkts/1(in_pol1_num_pkts) -> pipeline225/1(d)
  pol_tx_always_on/1(in_pol0_tx_always_on) -> pipeline217/1(d)
  pol_tx_always_on/2(in_pol1_tx_always_on) -> pipeline227/1(d)
  pol0_sample_offset/1(in_pol0_sample_offset) -> pipeline218/1(d)
  pol1_sample_offset/1(in_pol1_sample_offset) -> pipeline219/1(d)
  Delay87/1 -> pol_traffic_trigger/2(sim_2)
  pol_traffic_trigger/1(in_pol0_tx_trigger) -> pipeline222/1(d)
  pipeline221/1(q) -> Slice41/1
  Slice41/1 -> Convert4/1
  Convert4/1 -> [pol1_traffic_trigger]
  pol_traffic_trigger/2(in_pol1_tx_trigger) -> pipeline221/1(d)
  edge_detect31/1(out) -> Terminator66/1  "mrst"
  Constant170/1 -> freq_cwg0/1(sim_1)
  freq_cwg0/1(in_frequency) -> pipeline411/1(d)
  AddSub2/1 -> Slice21/1
  AddSub1/1 -> Slice22/1
  [tvg_stime] -> Gateway Out29/1, AddSub2/1, AddSub1/1
  Constant189/1 -> speadtime0_offset/1(sim_1)
  Slice21/1 -> Register5/1, Gateway Out13/1
  Slice22/1 -> Register6/1
  speadtime0_offset/1(in_speadtime_offset0) -> Gateway Out30/1, AddSub2/2
  Constant190/1 -> speadtime1_offset/1(sim_1)
  speadtime1_offset/1(in_speadtime_offset1) -> AddSub1/2
  Convert3/1 -> [pol0_traffic_trigger]
  Constant125/1 -> scale_cwg0/2(sim_2)
  Constant179/1 -> scale_cwg0/1(sim_1)
  Constant162/1 -> scale_out0/1(sim_1)
  Constant167/1 -> scale_out0/2(sim_2)
  scale_out0/2(in_dummy) -> Terminator15/1
  Constant164/1 -> Delay32/1
  Constant145/1 -> Delay87/1
  [cwg_80_1] -> pipeline290/1(d)
  [cwg_80_0] -> pipeline287/1(d)
  pipeline251/1(q) -> [source_sel_0]
  pipeline252/1(q) -> [source_sel_1]
  Constant194/1 -> src_sel_cntrl/1(sim_1)
  Constant195/1 -> src_sel_cntrl/2(sim_2)
  src_sel_cntrl/1(in_src_sel_0) -> pipeline251/1(d)
  src_sel_cntrl/2(in_src_sel_1) -> pipeline252/1(d)
  [source_sel_0] -> pipeline285/1(d)
  [source_sel_1] -> pipeline289/1(d)
  Mux9/1 -> pipeline292/1(d)
  Mux8/1 -> pipeline293/1(d)
  pipeline285/1(q) -> Mux9/1
  pipeline287/1(q) -> Mux9/2
  pipeline288/1(q) -> Mux9/3
  pipeline289/1(q) -> Mux8/1
  pipeline290/1(q) -> Mux8/2
  pipeline291/1(q) -> Mux8/3
  pipeline411/1(q) -> cwg0/1(freq)
  pipeline410/1(q) -> cwg0/2(scale)
  [mrst] -> pipeline276/1(d)
  Constant166/1 -> rpt_en_cwg0/2(sim_2)
  Constant168/1 -> rpt_length_cwg0/1(sim_1)
  rpt_en_cwg0/1(in_en) -> Convert25/1
  rpt_en_cwg0/2(in_dummy) -> Terminator71/1
  Constant177/1 -> rpt_en_cwg0/1(sim_1)
  Convert25/1 -> pipeline277/1(d)
  cwg0/1(bus_out) -> pipeline457/1(d), [Bus_expand_cwg0]
  rpt_length_cwg0/1(in_cwg0_repeat_length) -> pipeline278/1(d)
  pipeline276/1(q) -> cwg0/3(rst)
  pipeline277/1(q) -> cwg0/4(repeat_en)
  pipeline278/1(q) -> cwg0/5(repeat_length)
  [adc_count] -> Concat20/1
  Constant198/1 -> Concat20/2
  Delay73/1 -> [status0]
  Delay90/1 -> [status3]
  Delay89/1 -> [status2]
  Delay88/1 -> [status1]
  Concat20/1 -> Delay90/1, Delay73/1, Delay88/1, Delay89/1
  [ndiode_flag] -> Convert28/1
  Logical/1 -> Convert27/1
  Logical23/1 -> Convert30/1
  [adc_flag] -> Convert29/1
  [flag_en] -> Logical/1, Logical23/2
  Convert28/1 -> Logical/2
  Convert29/1 -> Logical23/1
  Convert30/1 -> Concat20/3
  Convert27/1 -> Concat20/4
  cwg0/3(rpt_rst) -> Terminator74/1
  pipeline257/1(q) -> Mux9/4
  [Impulse_gen0] -> pipeline257/1(d)
  pipeline258/1(q) -> Mux8/4
  [Impulse_gen0] -> pipeline258/1(d)
  pipeline417/1(q) -> bus_mult/1(a)
  Constant104/1 -> pipeline288/1(d)
  Constant105/1 -> pipeline291/1(d)
  pipeline292/1(q) -> Mux7/2
  Mux7/1 -> [data_80_0]
  [Start_Stop_Sel] -> Mux7/1
  Mux24/1 -> [data_80_1]
  pipeline293/1(q) -> Mux24/2
  Constant114/1 -> Mux24/3
  [Start_Stop_Sel] -> Mux24/1
  Constant115/1 -> Mux7/3
  Constant106/1 -> cwg0/6(en)
  pipeline457/1(q) -> bus_addsub2/1(a)
  edge_detect16/1(out) -> pipeline263/1(d)
  control1/4(in_cnt_rst) -> edge_detect14/1(in)
  edge_detect14/1(out) -> pipeline235/1(d)
  control1/3(in_gbe_rst) -> pipeline268/1(d)
  control1/1(in_sys_rst) -> pipeline246/1(d)
  pipeline246/1(q) -> [sys_rst]
  pipeline263/1(q) -> [clr_status]
  pipeline268/1(q) -> [gbe_rst]
  pipeline235/1(q) -> [cnt_rst]
  edge_detect15/1(out) -> pipeline249/1(d)
  pipeline249/1(q) -> [gbe_cnt_rst]
  control1/5(in_gbe_cnt_rst) -> edge_detect15/1(in)
  control1/2(in_status_clr) -> edge_detect16/1(in)
  cwg0/2(dvalid) -> Terminator42/1
  pipeline242/1(q) -> [gbe_port]
  scale_cwg0/1(in_scale) -> Gateway Out36/1, pipeline410/1(d)
  Gateway Out36/1 -> To Workspace228/1
  gbecontrol/1(in_gbe0) -> [gbe_txen0]
  gbecontrol/2(in_gbe1) -> [gbe_txen1]
  gbecontrol/3(in_gbe2) -> [gbe_txen2]
  gbecontrol/4(in_gbe3) -> [gbe_txen3]
  ramp0/1 -> [rampdata0]
  [vld0] -> ramp0/2
  [rdy0] -> ramp0/1
  ramp1/1 -> [rampdata1]
  [vld1] -> ramp1/2
  [rdy1] -> ramp1/1
  speadsnap_control/1(in_speadsnap_arm) -> Delay100/1
  Delay100/1 -> [speadsnap_arm]
  ramp2/1 -> [rampdata2]
  [vld2] -> ramp2/2
  [rdy2] -> ramp2/1
  ramp3/1 -> [rampdata3]
  [vld3] -> ramp3/2
  [rdy3] -> ramp3/1
  Constant116/1 -> gbecontrol/2(sim_2)
  Constant202/1 -> gbecontrol/1(sim_1)
  Constant117/1 -> gbecontrol/3(sim_3)
  Constant118/1 -> gbecontrol/4(sim_4)
  ramp80/1 -> [ramp79]
  [rst_ramp80] -> ramp80/1
  Delay102/1 -> [sel_ramp80]
  test_control/1(in_sel_ramp80) -> Delay102/1
  Delay103/1 -> [rst_ramp80]
  test_control/2(in_rst_ramp80) -> Delay103/1
  fifo4/1(fifo_data80) -> pipeline389/1(d)  "data00"
  fifo4/2(fifo_dv) -> pipeline390/1(d)  "dv00"
  fifo4/3(word_start) -> pipeline391/1(d)  "ws00"
  fifo4/4(pkt_start) -> pipeline392/1(d)  "ps00"
  fifo4/5(fifo_full) -> Terminator40/1  "full00"
  fifo4/6(fifo_empty) -> Terminator56/1  "empty00"
  fifo5/1(fifo_data80) -> pipeline430/1(d)  "data01"
  fifo5/2(fifo_dv) -> pipeline431/1(d)  "dv01"
  fifo5/3(word_start) -> pipeline432/1(d)  "ws01"
  fifo5/4(pkt_start) -> pipeline433/1(d)  "ps01"
  pack_80_64_5/2(valid64) -> pipeline449/1(d)  "v64_01"
  pack_80_64_5/1(ready64) -> pipeline448/1(d)  "r64_01"
  fifo5/5(fifo_full) -> Terminator41/1
  fifo5/6(fifo_empty) -> Terminator54/1
  [hdr_0x3101] -> bus_create10/1(in1)
  [pol0_id] -> bus_create10/2(in2)
  [hdr_0x3101] -> bus_create4/1(in1)
  [pol0_id] -> bus_create4/2(in2)
  [speadtime0] -> Gateway Out44/1, spead_pack4/8(hdr5_0x1600_DIR), spead_pack4/4(hdr_heap_id)  "timein0"
  bus_create10/1(bus_out) -> spead_pack4/9(hdr6_0x3101_DIR)
  [status0] -> spead_pack4/10(hdr7_0x3102_DIR)
  bus_create4/1(bus_out) -> spead_pack5/9(hdr6_0x3101_DIR)
  [status1] -> spead_pack5/10(hdr7_0x3102_DIR)
  [tvg_ltime] -> fifo_select1/1(localtime)
  fifo_select1/1(fifo_select0) -> fifo4/2(fifo_we_en), Gateway Out15/1, [fifoselect]  "fifoselect0"
  [speadtime1] -> spead_pack5/4(hdr_heap_id), spead_pack5/8(hdr5_0x1600_DIR)  "timein1"
  pack_80_64_4/1(ready64) -> pipeline446/1(d)  "r64_00"
  pack_80_64_4/2(valid64) -> pipeline447/1(d)  "v64_00"
  [spead_heapsize] -> spead_pack4/5(hdr_heap_size)
  [spead_heapoffset] -> spead_pack4/6(hdr_heap_offset)
  [spead_pktlen] -> spead_pack4/7(hdr_pkt_len_words)
  [spead_heapsize] -> spead_pack5/5(hdr_heap_size)
  [spead_heapoffset] -> spead_pack5/6(hdr_heap_offset)
  [spead_pktlen] -> spead_pack5/7(hdr_pkt_len_words)
  spead_pack5/4(data_overflow) -> Terminator39/1
  [adc_data_offset] -> spead_pack4/11(hdr8_0x3300)
  [adc_data_offset] -> spead_pack5/11(hdr8_0x3300)
  Constant121/1 -> [spead_heapsize]
  Constant122/1 -> [spead_pktlen]
  Constant126/1 -> [spead_heapoffset]
  spead_pack4/4(data_overflow) -> Terminator38/1
  spead_pack4/3(eof) -> pipeline334/1(d)
  spead_pack4/1(data_out) -> pipeline330/1(d)  "packd"
  spead_pack4/2(valid_out) -> pipeline333/1(d)  "packv"
  spead_pack5/1(data_out) -> pipeline340/1(d)
  spead_pack5/2(valid_out) -> pipeline341/1(d)
  spead_pack5/3(eof) -> pipeline342/1(d)
  Constant141/1 -> [adc_data_offset]
  pipeline330/1(q) -> [spead_data0]
  pipeline333/1(q) -> Gateway Out55/1, [spead_valid0]  "sp_dv0"
  pipeline334/1(q) -> [spead_eof0]
  pipeline340/1(q) -> [spead_data1]
  pipeline341/1(q) -> Gateway Out56/1, [spead_valid1]  "sp_dv1"
  pipeline342/1(q) -> [spead_eof1]
  pipeline389/1(q) -> Gateway Out18/1, Mux12/2  "d80"
  pipeline390/1(q) -> pack_80_64_4/2(valid80)  "v80"
  pipeline391/1(q) -> pack_80_64_4/3(word_start)  "wd_start"
  pipeline392/1(q) -> Delay109/1, pack_80_64_4/4(pkt_start)  "pkt_start"
  pipeline430/1(q) -> Mux13/2
  pipeline431/1(q) -> pack_80_64_5/2(valid80)
  pipeline432/1(q) -> pack_80_64_5/3(word_start)
  pipeline433/1(q) -> Delay113/1, pack_80_64_5/4(pkt_start)
  pipeline447/1(q) -> [vld0], spead_pack4/2(data64_valid)
  pipeline448/1(q) -> [rdy1], spead_pack5/1(data64_ready)  "rdy1"
  pipeline449/1(q) -> [vld1], spead_pack5/2(data64_valid)
  fifo_select1/2(fifo_select1) -> Gateway Out16/1, fifo5/2(fifo_we_en)  "fifoselect1"
  Mux20/1 -> Gateway Out43/1, spead_pack4/3(data64)
  Mux21/1 -> spead_pack5/3(data64)
  [spead_data0] -> pipeline451/1(d)
  [spead_valid0] -> pipeline452/1(d)
  wr_addr0/1 -> 64_to_256/1  "waddr"
  [spead_valid0] -> edge_detect28/1(in), edge_detect39/1, pipeline450/1(d)
  Constant129/1 -> 64_to_256/6
  Constant130/1 -> 64_to_256/5
  rd_addr0/1 -> 64_to_256/4, Relational23/2  "rdaddr"
  64_to_256/2 -> pipeline270/1(d)
  edge_detect39/1 -> wr_addr0/1
  pipeline450/1(q) -> wr_addr0/2
  pipeline451/1(q) -> 64_to_256/2
  pipeline452/1(q) -> 64_to_256/3  "dv64_0"
  64_to_256/1 -> Terminator61/1
  edge_detect28/1(out) -> rd_addr0/1, rd_arm/3, rd_arm/1
  Constant140/1 -> Relational23/1
  Relational23/1 -> rd_arm/2  "rd_done"
  rd_arm/1 -> pipeline453/1(d), 64_to_256/7, rd_addr0/2  "rd_en"
  pipeline453/1(q) -> edge_detect8/1(in), pipeline223/1(d)
  edge_detect8/1(out) -> [sp256_eof0]  "eof256_0"
  fifo6/1(fifo_data80) -> pipeline348/1(d)  "data00"
  fifo6/2(fifo_dv) -> pipeline349/1(d)  "dv00"
  fifo6/3(word_start) -> pipeline351/1(d)  "ws00"
  fifo6/4(pkt_start) -> pipeline352/1(d)  "ps00"
  fifo6/5(fifo_full) -> Terminator57/1  "full00"
  fifo6/6(fifo_empty) -> Terminator60/1  "empty00"
  fifo7/1(fifo_data80) -> pipeline271/1(d)  "data01"
  fifo7/2(fifo_dv) -> pipeline272/1(d)  "dv01"
  fifo7/3(word_start) -> pipeline273/1(d)  "ws01"
  fifo7/4(pkt_start) -> pipeline274/1(d)  "ps01"
  pack_80_64_7/2(valid64) -> pipeline328/1(d)  "v64_01"
  pack_80_64_7/1(ready64) -> pipeline327/1(d)  "r64_01"
  fifo7/5(fifo_full) -> Terminator58/1
  fifo7/6(fifo_empty) -> Terminator59/1
  [hdr_0x3101] -> bus_create6/1(in1)
  [pol1_id] -> bus_create6/2(in2)
  [hdr_0x3101] -> bus_create5/1(in1)
  [pol1_id] -> bus_create5/2(in2)
  [speadtime0] -> spead_pack6/4(hdr_heap_id), spead_pack6/8(hdr5_0x1600_DIR)  "timein0"
  bus_create6/1(bus_out) -> spead_pack6/9(hdr6_0x3101_DIR)
  [status2] -> spead_pack6/10(hdr7_0x3102_DIR)
  bus_create5/1(bus_out) -> spead_pack7/9(hdr6_0x3101_DIR)
  [status3] -> spead_pack7/10(hdr7_0x3102_DIR)
  fifo_select2/1(fifo_select0) -> fifo6/2(fifo_we_en)  "fifoselect2"
  [speadtime1] -> spead_pack7/8(hdr5_0x1600_DIR), spead_pack7/4(hdr_heap_id)  "timein1"
  pack_80_64_6/1(ready64) -> pipeline294/1(d)  "r64_00"
  pack_80_64_6/2(valid64) -> pipeline307/1(d)  "v64_00"
  [spead_heapsize] -> spead_pack6/5(hdr_heap_size)
  [spead_heapoffset] -> spead_pack6/6(hdr_heap_offset)
  [spead_pktlen] -> spead_pack6/7(hdr_pkt_len_words)
  [spead_heapsize] -> spead_pack7/5(hdr_heap_size)
  [spead_heapoffset] -> spead_pack7/6(hdr_heap_offset)
  [spead_pktlen] -> spead_pack7/7(hdr_pkt_len_words)
  Assert3/1 -> fifo6/1(data80), fifo7/1(data80)
  spead_pack7/4(data_overflow) -> Terminator53/1
  [adc_data_offset] -> spead_pack6/11(hdr8_0x3300)
  [adc_data_offset] -> spead_pack7/11(hdr8_0x3300)
  spead_pack6/4(data_overflow) -> Terminator79/1
  spead_pack6/3(eof) -> pipeline344/1(d)
  spead_pack6/1(data_out) -> pipeline329/1(d)  "packd"
  spead_pack6/2(valid_out) -> pipeline343/1(d)  "packv"
  spead_pack7/1(data_out) -> pipeline345/1(d)
  spead_pack7/2(valid_out) -> pipeline346/1(d)
  spead_pack7/3(eof) -> pipeline347/1(d)
  pipeline329/1(q) -> [spead_data2]
  pipeline343/1(q) -> Gateway Out57/1, [spead_valid2]  "sp_dv0"
  pipeline344/1(q) -> [spead_eof2]
  pipeline345/1(q) -> [spead_data3]
  pipeline346/1(q) -> Gateway Out58/1, [spead_valid3]  "sp_dv1"
  pipeline347/1(q) -> [spead_eof3]
  pipeline349/1(q) -> pack_80_64_6/2(valid80)
  pipeline351/1(q) -> pack_80_64_6/3(word_start)
  pipeline352/1(q) -> Delay117/1, pack_80_64_6/4(pkt_start)
  pipeline272/1(q) -> pack_80_64_7/2(valid80)
  pipeline273/1(q) -> pack_80_64_7/3(word_start)
  pipeline274/1(q) -> Delay104/1, pack_80_64_7/4(pkt_start)
  pipeline294/1(q) -> spead_pack6/1(data64_ready), [rdy2]  "rdy2"
  pipeline307/1(q) -> spead_pack6/2(data64_valid), [vld2]
  pipeline327/1(q) -> spead_pack7/1(data64_ready), [rdy3]  "rdy3"
  pipeline328/1(q) -> spead_pack7/2(data64_valid), [vld3]
  fifo_select2/2(fifo_select1) -> fifo7/2(fifo_we_en)  "fifoselect3"
  Mux11/1 -> spead_pack7/3(data64)
  [spead_data2] -> pipeline354/1(d)
  [spead_valid2] -> pipeline355/1(d)
  wr_addr2/1 -> 64_to_1/1  "waddr"
  [spead_valid2] -> pipeline353/1(d), edge_detect18/1, edge_detect21/1(in)
  Constant119/1 -> 64_to_1/6
  Constant120/1 -> 64_to_1/5
  rd_addr2/1 -> Relational13/2, 64_to_1/4  "rdaddr"
  64_to_1/2 -> pipeline365/1(d)
  edge_detect18/1 -> wr_addr2/1
  pipeline353/1(q) -> wr_addr2/2
  pipeline354/1(q) -> 64_to_1/2
  pipeline355/1(q) -> 64_to_1/3  "dv64_2"
  64_to_1/1 -> Terminator62/1
  edge_detect21/1(out) -> rd_addr2/1
  Constant128/1 -> Relational13/1
  Relational13/1 -> rd_arm2/2  "rd_done"
  rd_arm2/1 -> 64_to_1/7, rd_addr2/2, pipeline356/1(d)  "rd_en"
  pipeline356/1(q) -> edge_detect19/1(in), pipeline364/1(d)  "dv256"
  edge_detect19/1(out) -> [sp256_eof2]  "eof256_2"
  pipeline364/1(q) -> [sp256_dv2]  "dv256_2"
  [sp256_eof0] -> rd_arm2/3, rd_arm2/1
  [spead_data1] -> pipeline367/1(d)
  [spead_valid1] -> pipeline368/1(d)
  wr_addr1/1 -> 64_to_2/1  "waddr"
  [spead_valid1] -> pipeline366/1(d), edge_detect22/1, edge_detect24/1(in)
  Constant131/1 -> 64_to_2/6
  Constant132/1 -> 64_to_2/5
  rd_addr1/1 -> Relational6/2, 64_to_2/4  "rdaddr"
  64_to_2/2 -> pipeline371/1(d)
  edge_detect22/1 -> wr_addr1/1
  pipeline366/1(q) -> wr_addr1/2
  pipeline367/1(q) -> 64_to_2/2
  pipeline368/1(q) -> 64_to_2/3  "dv64_1"
  64_to_2/1 -> Terminator63/1
  edge_detect24/1(out) -> rd_arm1/3, rd_arm1/1, rd_addr1/1
  Constant133/1 -> Relational6/1
  Relational6/1 -> rd_arm1/2  "rd_done"
  rd_arm1/1 -> 64_to_2/7, rd_addr1/2, pipeline369/1(d)  "rd_en"
  pipeline369/1(q) -> pipeline370/1(d), edge_detect23/1(in)  "dv256"
  edge_detect23/1(out) -> [sp256_eof1]  "eof256_1"
  pipeline370/1(q) -> [sp256_dv1]  "dv256_1"
  [spead_data3] -> pipeline374/1(d)
  [spead_valid3] -> pipeline375/1(d)
  wr_addr3/1 -> 64_to_3/1  "waddr"
  [spead_valid3] -> edge_detect27/1(in), edge_detect25/1, pipeline373/1(d)
  Constant134/1 -> 64_to_3/6
  Constant135/1 -> 64_to_3/5
  rd_addr3/1 -> 64_to_3/4, Relational11/2  "rdaddr"
  64_to_3/2 -> pipeline378/1(d)
  edge_detect25/1 -> wr_addr3/1
  pipeline373/1(q) -> wr_addr3/2
  pipeline374/1(q) -> 64_to_3/2
  pipeline375/1(q) -> 64_to_3/3  "dv64_3"
  64_to_3/1 -> Terminator81/1
  edge_detect27/1(out) -> rd_addr3/1
  Constant136/1 -> Relational11/1
  Relational11/1 -> rd_arm3/2  "rd_done"
  rd_arm3/1 -> pipeline376/1(d), 64_to_3/7, rd_addr3/2  "rd_en"
  pipeline376/1(q) -> edge_detect26/1(in), pipeline377/1(d)  "dv256"
  edge_detect26/1(out) -> [sp256_eof3]  "eof256_3"
  pipeline377/1(q) -> [sp256_dv3]  "dv256_3"
  [sp256_eof1] -> rd_arm3/1, rd_arm3/3
  [sp256_dv0] -> Mux6/1  "dv0"
  [sp256_data0] -> Mux6/3
  [sp256_data2] -> Mux6/2
  [sp256_dv1] -> pipeline436/1(d)  "dv1"
  Mux6/1 -> Mux25/2
  [sp256_data1] -> pipeline379/1(d)
  [sp256_dv3] -> pipeline437/1(d)  "dv3"
  Mux25/1 -> Mux26/2
  [sp256_data3] -> pipeline380/1(d)
  Mux26/1 -> Gateway Out53/1, munge/1(din)
  pipeline379/1(q) -> Mux25/3
  pipeline380/1(q) -> pipeline381/1(d)
  pipeline381/1(q) -> Mux26/3
  [sp256_dvg0] -> Logical39/1
  [sp256_dvg1] -> Logical39/2
  [sp256_dvg2] -> Logical39/3
  [sp256_dvg3] -> Logical39/4
  Logical39/1 -> pipeline386/1(d)
  pipeline386/1(q) -> pipeline387/1(d)
  pipeline387/1(q) -> [sp256_dv]
  [sp256_eofg0] -> Logical8/1
  [sp256_eofg1] -> Logical8/2
  [sp256_eofg2] -> Logical8/3
  [sp256_eofg3] -> Logical8/4
  Logical8/1 -> pipeline388/1(d)
  pipeline388/1(q) -> pipeline435/1(d)
  pipeline435/1(q) -> [sp256_eof]  "tx_eof"
  [sp256_dv0] -> Mux17/1
  [gbe_ip2] -> Mux17/2
  [sp256_dv1] -> pipeline421/1(d)
  Mux17/1 -> Mux18/2
  [gbe_ip1] -> pipeline382/1(d)
  [sp256_dv3] -> pipeline422/1(d)
  Mux18/1 -> Mux19/2
  [gbe_ip3] -> pipeline384/1(d)
  Mux19/1 -> [gbe_txip]
  pipeline382/1(q) -> Mux18/3
  pipeline384/1(q) -> pipeline385/1(d)
  pipeline385/1(q) -> Mux19/3
  [gbe_txen0] -> Logical9/2
  pipeline223/1(q) -> [sp256_dv0]  "dv256_0"
  [sp256_eof0] -> Logical9/1
  [sp256_dv0] -> Logical13/1
  [gbe_txen0] -> Logical13/2
  Logical13/1 -> Gateway Out46/1, [sp256_dvg0]
  Logical9/1 -> Gateway Out45/1, [sp256_eofg0]
  [gbe_txen1] -> Logical17/2
  [sp256_eof1] -> Logical17/1
  [sp256_dv1] -> Logical18/1
  [gbe_txen1] -> Logical18/2
  Logical18/1 -> Gateway Out48/1, [sp256_dvg1]
  Logical17/1 -> Gateway Out47/1, [sp256_eofg1]
  [gbe_txen2] -> Logical19/2
  [sp256_eof2] -> Logical19/1
  [sp256_dv2] -> Logical20/1
  [gbe_txen2] -> Logical20/2
  Logical20/1 -> Gateway Out50/1, [sp256_dvg2]
  Logical19/1 -> Gateway Out49/1, [sp256_eofg2]
  [gbe_txen3] -> Logical47/2
  [sp256_eof3] -> Logical47/1
  [sp256_dv3] -> Logical22/1
  [gbe_txen3] -> Logical22/2
  Logical22/1 -> Gateway Out52/1, [sp256_dvg3]
  Logical47/1 -> Gateway Out51/1, [sp256_eofg3]
  pipeline436/1(q) -> Mux25/1  "msel2"
  pipeline437/1(q) -> pipeline438/1(d)
  pipeline438/1(q) -> Mux26/1  "msel3"
  [rampdata0] -> Mux20/2
  [sel_ramp80] -> Mux20/1
  pack_80_64_4/3(data64) -> pipeline439/1(d)
  pipeline439/1(q) -> Mux20/3
  [rampdata1] -> Mux21/2
  [sel_ramp80] -> Mux21/1
  pipeline440/1(q) -> Mux21/3
  pack_80_64_5/3(data64) -> pipeline440/1(d)  "d64_00"
  [rampdata2] -> Mux10/2
  [sel_ramp80] -> Mux10/1
  pipeline441/1(q) -> Mux10/3
  [rampdata3] -> Mux11/2
  [sel_ramp80] -> Mux11/1
  pipeline442/1(q) -> Mux11/3
  pack_80_64_7/3(data64) -> pipeline442/1(d)
  pack_80_64_6/3(data64) -> pipeline441/1(d)
  Mux10/1 -> spead_pack6/3(data64)
  [speadtime0] -> Gateway Out19/1, Mux12/3
  Mux12/1 -> Gateway Out20/1, [data_80_tp], pack_80_64_4/1(data80)  "d80_in"
  Delay113/1 -> Mux13/1
  [speadtime1] -> Mux13/3
  Mux13/1 -> pack_80_64_5/1(data80)
  Delay117/1 -> Mux14/1
  [speadtime0] -> Mux14/3
  Mux14/1 -> pack_80_64_6/1(data80)
  pipeline348/1(q) -> Mux14/2
  Delay104/1 -> Mux15/1
  [speadtime1] -> Mux15/3
  Mux15/1 -> pack_80_64_7/1(data80)
  pipeline271/1(q) -> Mux15/2
  [tvg_select0] -> Delay118/1
  Delay118/1 -> Mux22/1
  Delay119/1 -> Mux22/2
  Delay125/1 -> Mux22/3
  [tvg_pol0] -> Delay119/1
  [data_80_0] -> Delay125/1
  Mux22/1 -> Assert2/1
  [tvg_select1] -> Delay135/1
  Mux23/1 -> Assert3/1  "d80_0"
  [data_80_1] -> Delay137/1
  [tvg_pol1] -> Delay136/1
  Delay135/1 -> Mux23/1
  Delay137/1 -> Mux23/3
  Delay136/1 -> Mux23/2
  [gbe_ip0] -> Mux17/3
  pipeline421/1(q) -> Mux18/1
  pipeline422/1(q) -> Mux19/1
  Assert2/1 -> fifo5/1(data80), fifo4/1(data80)
  [mrst] -> fifo_select1/2(rst)
  [tvg_ltime] -> fifo_select2/1(localtime)
  [mrst] -> fifo_select2/2(rst)
  Constant87/1 -> test_control/1(sim_1)
  Constant91/1 -> test_control/2(sim_2)
  Gateway Out213/1 -> To Workspace213/1
  [speadtime0] -> Gateway Out213/1
  Gateway Out221/1 -> To Workspace221/1
  [speadtime1] -> Gateway Out221/1
  bus_constant/1(dout) -> pipeline458/1(d)
  unpack_and_reorder/5(recvd) -> Gateway Out11/1, ts_tvg/6(recvd_in)
  sync_gen/2(dout) -> bus_expand6/1(bus_in)
  sync_gen/3(dvalid) -> impulse_gen0/6(en), impulse_gen1/6(en)
  Slice12/1 -> [time80], Gateway Out86/1
  impulse_gen0/3(dvalid) -> Gateway Out12/1, [valid80]
  impulse_gen0/2(dout) -> [d80_adc0]
  impulse_gen0/4(misco) -> [time80_48], Gateway Out87/1, Slice12/1
  [tvg_adc0_en] -> impulse_gen0/1(tvg_en)
  impulse_gen1/1(sync_out) -> Terminator6/1
  impulse_gen1/2(dout) -> [d80_adc1]
  impulse_gen1/3(dvalid) -> Terminator8/1
  impulse_gen1/4(misco) -> [dig_flags]
  [tvg_adc1_en] -> impulse_gen1/1(tvg_en)
  impulse0/1(in_offset) -> Slice7/1
  impulse0/2(in_amplitude) -> impulse_gen0/3(impulse_amplitude)
  impulse1/1(in_offset) -> Slice8/1
  impulse1/2(in_amplitude) -> impulse_gen1/3(impulse_amplitude)
  sync_gen/1(sync) -> impulse_gen0/4(sync_in), impulse_gen1/4(sync_in)
  bus_expand6/1(msb_out2) -> bus_expand/1(bus_in), impulse_gen0/5(din)
  bus_expand6/2(lsb_out1) -> impulse_gen1/5(din)
  sync_gen/5(misco) -> impulse_gen1/7(misci)
  sync_gen/4(time_out) -> Gateway Out89/1, impulse_gen0/7(misci)
  Constant31/1 -> Concat9/2
  Logical15/1 -> edge_detect17/1(in)
  edge_detect17/1(out) -> [sys_relock]
  Concat9/1 -> Gateway Out88/1, sync_gen/1(time_in)
  [sys_relock] -> sync_gen/5(relock)
  [unpack_dv] -> sync_gen/2(en)
  [unpack_d160] -> bus_expand2/1(bus_in), sync_gen/3(din)
  Slice7/1 -> impulse_gen0/2(impulse_offset)
  Slice8/1 -> impulse_gen1/2(impulse_offset)
  edge_detect4/1(out) -> pipeline5/1(d)
  control/7(in_cnt_rst) -> edge_detect1/1(in)
  edge_detect1/1(out) -> pipeline14/1(d)
  control/3(in_gbe_rst) -> pipeline6/1(d)
  control/1(in_sys_rst) -> pipeline3/1(d)
  pipeline3/1(q) -> Terminator86/1
  pipeline5/1(q) -> Terminator87/1
  pipeline6/1(q) -> Terminator88/1
  pipeline7/1(q) -> [gbe_txen]
  pipeline13/1(q) -> [tvg_adc0_en]
  pipeline14/1(q) -> Terminator89/1
  control/5(in_tvg_adc0) -> pipeline13/1(d)
  edge_detect2/1(out) -> pipeline38/1(d)
  pipeline38/1(q) -> Terminator90/1
  control/8(in_gbe_cnt_rst) -> edge_detect2/1(in)
  control/4(in_gbe_txen) -> pipeline7/1(d)
  control/2(in_status_clr) -> edge_detect4/1(in)
  pipeline43/1(q) -> [adc_snap_arm]
  control/9(in_adc_snap_arm) -> pipeline43/1(d)
  control/10(in_adc_snap_trig_select) -> pipeline39/1(d)
  pipeline39/1(q) -> [adc_snap_trig_source]
  unpack_and_reorder/3(dv) -> Gateway Out9/1, ts_tvg/4(dv_in)
  unpack_and_reorder/4(time) -> Gateway Out10/1, ts_tvg/5(time_in)
  unpack_and_reorder/1(sync) -> Gateway Out6/1, ts_tvg/2(sync_in)
